simulink model "IRB140"  (R2016b)
settings: Solver=ode113  StartTime=0.0  StopTime=40  RelTol=1e-3
(part 6 of 9)

== matlab function IRB140/Robot2 ==
  data: u input; thetadd output; theta input; thetad input; D output; V output; G output
function [thetadd, D, V, G] = fcn(u, theta, thetad)
theta1 = theta(1);
theta2 = theta(2);
theta3 = theta(3);
theta4 = theta(4);
theta5 = theta(5);
theta6 = theta(6);

qd1 = thetad(1);
qd2 = thetad(2);
qd3 = thetad(3);
qd4 = thetad(4);
qd5 = thetad(5);
qd6 = thetad(6);

g = 9.81;

G1 = 0;
G2 = (g*(57*sin(theta2)*cos(theta3)*cos(theta4)*sin(theta5) + 57*sin(theta3)*cos(theta2)*cos(theta4)*sin(theta5) ...
    + 57*sin(theta2)*sin(theta3)*cos(theta5) + 3186*sin(theta2)*cos(theta3)*sin(theta4) ... 
    + 3186*sin(theta3)*cos(theta2)*sin(theta4) - 57*cos(theta2)*cos(theta3)*cos(theta5) + 418*sin(theta2)*sin(theta3) ... 
    - 418*cos(theta2)*cos(theta3) - 99072*sin(theta2)))/20000;
G3 = 57*(((-cos(theta5) - 22/3)*cos(theta3) + (1062*sin(theta3)*((19*cos(theta4)*sin(theta5))/1062 ...
    + sin(theta4)))/19)*cos(theta2) + ((cos(theta4)*sin(theta5) + (1062*sin(theta4))/19)*cos(theta3) ...
    + (cos(theta5) + 22/3)*sin(theta3))*sin(theta2))*g/20000;
G4 = -57*(sin(theta2)*sin(theta3) - cos(theta2)*cos(theta3))*g*(sin(theta4)*sin(theta5) - (1062*cos(theta4))/19)/20000;
G5 = 57*(cos(theta5)*(sin(theta2)*sin(theta3) - cos(theta2)*cos(theta3))*cos(theta4) ...
    + (cos(theta2)*sin(theta3) + sin(theta2)*cos(theta3))*sin(theta5))*g/20000;
G6 = 0;

G = [G1; G2; G3; G4; G5; G6];

d11 = (19271109*cos(2*theta5))/8000000000 - (386153977*cos(2*theta4))/8000000000 - (295248399*cos(2*theta2))/400000000 - (814991*cos(2*theta6))/2000000000 + (8551647*sin(2*theta2))/200000000 + (510879*sin(2*theta4))/1000000000 + (5043*sin(2*theta5))/500000000 - (1083*cos(theta5))/1000000 - (10836*sin(theta2))/15625 - (1881*sin(theta3))/250000 - (1463*cos(theta2)*cos(theta3))/500000 - (14337*cos(theta3)*sin(theta4))/250000 - (513*cos(theta5)*sin(theta3))/500000 + (1463*sin(theta2)*sin(theta3))/500000 + (1881*cos(2*theta2)*sin(theta3))/250000 + (1881*sin(2*theta2)*cos(theta3))/250000 - (46480089*sin(2*theta4)*cos(theta5))/2000000000 - (2310763*sin(2*theta5)*cos(theta6))/1000000000 + (63931*sin(2*theta4)*sin(theta5))/2000000000 + (3685180549*cos(2*theta2)*cos(2*theta3))/8000000000 - (19271109*cos(2*theta4)*cos(2*theta5))/8000000000 - (2444973*cos(2*theta4)*cos(2*theta6))/2000000000 + (814991*cos(2*theta5)*cos(2*theta6))/2000000000 - (2389617*cos(2*theta2)*sin(2*theta3))/1000000000 - (2389617*cos(2*theta3)*sin(2*theta2))/1000000000 - (5043*cos(2*theta4)*sin(2*theta5))/500000000 - (3685180549*sin(2*theta2)*sin(2*theta3))/8000000000 - (386153977*cos(2*theta2)*cos(2*theta3)*cos(2*theta4))/8000000000 - (57813327*cos(2*theta2)*cos(2*theta3)*cos(2*theta5))/8000000000 + (2444973*cos(2*theta2)*cos(2*theta3)*cos(2*theta6))/2000000000 - (814991*cos(2*theta4)*cos(2*theta5)*cos(2*theta6))/2000000000 + (11151*cos(theta2)*sin(theta3)*sin(theta4))/500000 + (11151*cos(theta3)*sin(theta2)*sin(theta4))/500000 + (399*cos(theta5)*sin(theta2)*sin(theta3))/1000000 + (510879*cos(2*theta2)*cos(2*theta3)*sin(2*theta4))/1000000000 - (15129*cos(2*theta2)*cos(2*theta3)*sin(2*theta5))/500000000 + (386153977*cos(2*theta4)*sin(2*theta2)*sin(2*theta3))/8000000000 + (57813327*cos(2*theta5)*sin(2*theta2)*sin(2*theta3))/8000000000 - (2444973*cos(2*theta6)*sin(2*theta2)*sin(2*theta3))/2000000000 - (510879*sin(2*theta2)*sin(2*theta3)*sin(2*theta4))/1000000000 + (15129*sin(2*theta2)*sin(2*theta3)*sin(2*theta5))/500000000 + (14337*cos(2*theta2)*cos(theta3)*sin(theta4))/250000 + (513*cos(2*theta2)*cos(theta5)*sin(theta3))/500000 + (513*sin(2*theta2)*cos(theta3)*cos(theta5))/500000 - (14337*sin(2*theta2)*sin(theta3)*sin(theta4))/250000 - (2310763*sin(2*theta4)*sin(theta5)*sin(theta6))/500000000 - (1083*cos(2*theta2)*cos(2*theta3)*cos(theta5))/1000000 + (240014043*cos(2*theta2)*sin(2*theta3)*cos(theta4))/500000000 + (240014043*cos(2*theta3)*sin(2*theta2)*cos(theta4))/500000000 + (2310763*cos(2*theta4)*sin(2*theta5)*cos(theta6))/1000000000 + (58876307*cos(2*theta2)*sin(2*theta3)*sin(theta4))/1000000000 + (58876307*cos(2*theta3)*sin(2*theta2)*sin(theta4))/1000000000 + (1083*sin(2*theta2)*sin(2*theta3)*cos(theta5))/1000000 + (814991*sin(2*theta4)*sin(2*theta6)*cos(theta5))/500000000 - (399*cos(theta2)*cos(theta3)*cos(theta5))/1000000 - (513*cos(theta3)*cos(theta4)*sin(theta5))/500000 + (46480089*sin(2*theta2)*sin(2*theta3)*sin(2*theta4)*cos(theta5))/2000000000 - (6932289*sin(2*theta2)*sin(2*theta3)*sin(2*theta5)*cos(theta6))/1000000000 - (63931*sin(2*theta2)*sin(2*theta3)*sin(2*theta4)*sin(theta5))/2000000000 + (513*cos(2*theta2)*cos(theta3)*cos(theta4)*sin(theta5))/500000 - (19271109*cos(2*theta2)*cos(2*theta3)*cos(2*theta4)*cos(2*theta5))/8000000000 - (2444973*cos(2*theta2)*cos(2*theta3)*cos(2*theta4)*cos(2*theta6))/2000000000 - (2444973*cos(2*theta2)*cos(2*theta3)*cos(2*theta5)*cos(2*theta6))/2000000000 - (5043*cos(2*theta2)*cos(2*theta3)*cos(2*theta4)*sin(2*theta5))/500000000 - (513*sin(2*theta2)*cos(theta4)*sin(theta3)*sin(theta5))/500000 + (19271109*cos(2*theta4)*cos(2*theta5)*sin(2*theta2)*sin(2*theta3))/8000000000 + (2444973*cos(2*theta4)*cos(2*theta6)*sin(2*theta2)*sin(2*theta3))/2000000000 + (2444973*cos(2*theta5)*cos(2*theta6)*sin(2*theta2)*sin(2*theta3))/2000000000 + (5043*cos(2*theta4)*sin(2*theta2)*sin(2*theta3)*sin(2*theta5))/500000000 + (1083*cos(2*theta2)*sin(2*theta3)*cos(theta4)*sin(theta5))/1000000 + (63931*cos(2*theta2)*sin(2*theta3)*cos(theta5)*sin(theta4))/1000000000 + (1083*cos(2*theta3)*sin(2*theta2)*cos(theta4)*sin(theta5))/1000000 + (63931*cos(2*theta3)*sin(2*theta2)*cos(theta5)*sin(theta4))/1000000000 + (46480089*cos(2*theta2)*sin(2*theta3)*sin(theta4)*sin(theta5))/1000000000 + (46480089*cos(2*theta3)*sin(2*theta2)*sin(theta4)*sin(theta5))/1000000000 + (399*cos(theta2)*cos(theta4)*sin(theta3)*sin(theta5))/1000000 + (399*cos(theta3)*cos(theta4)*sin(theta2)*sin(theta5))/1000000 - (46480089*cos(2*theta2)*cos(2*theta3)*sin(2*theta4)*cos(theta5))/2000000000 - (5043*cos(2*theta2)*cos(2*theta5)*sin(2*theta3)*cos(theta4))/125000000 - (5043*cos(2*theta3)*cos(2*theta5)*sin(2*theta2)*cos(theta4))/125000000 + (6932289*cos(2*theta2)*cos(2*theta3)*sin(2*theta5)*cos(theta6))/1000000000 + (63931*cos(2*theta2)*cos(2*theta3)*sin(2*theta4)*sin(theta5))/2000000000 + (19271109*cos(2*theta2)*sin(2*theta3)*sin(2*theta5)*cos(theta4))/2000000000 + (19271109*cos(2*theta3)*sin(2*theta2)*sin(2*theta5)*cos(theta4))/2000000000 + (2310763*sin(2*theta2)*sin(2*theta3)*sin(2*theta4)*sin(theta5)*sin(theta6))/500000000 + (2310763*cos(2*theta2)*cos(2*theta3)*cos(2*theta4)*sin(2*theta5)*cos(theta6))/1000000000 + (814991*cos(2*theta2)*cos(2*theta3)*sin(2*theta4)*sin(2*theta6)*cos(theta5))/500000000 + (814991*cos(2*theta2)*cos(2*theta6)*sin(2*theta3)*sin(2*theta5)*cos(theta4))/500000000 + (814991*cos(2*theta3)*cos(2*theta6)*sin(2*theta2)*sin(2*theta5)*cos(theta4))/500000000 - (2310763*cos(2*theta4)*sin(2*theta2)*sin(2*theta3)*sin(2*theta5)*cos(theta6))/1000000000 - (814991*sin(2*theta2)*sin(2*theta3)*sin(2*theta4)*sin(2*theta6)*cos(theta5))/500000000 - (814991*cos(2*theta2)*cos(2*theta3)*cos(2*theta4)*cos(2*theta5)*cos(2*theta6))/2000000000 - (2310763*cos(2*theta2)*sin(2*theta3)*cos(theta5)*sin(theta4)*sin(theta6))/250000000 - (2310763*cos(2*theta3)*sin(2*theta2)*cos(theta5)*sin(theta4)*sin(theta6))/250000000 + (814991*cos(2*theta4)*cos(2*theta5)*cos(2*theta6)*sin(2*theta2)*sin(2*theta3))/2000000000 + (2310763*cos(2*theta2)*cos(2*theta5)*sin(2*theta3)*cos(theta4)*cos(theta6))/250000000 + (2310763*cos(2*theta3)*cos(2*theta5)*sin(2*theta2)*cos(theta4)*cos(theta6))/250000000 - (2310763*cos(2*theta2)*cos(2*theta3)*sin(2*theta4)*sin(theta5)*sin(theta6))/500000000 - (814991*cos(2*theta2)*sin(2*theta3)*sin(2*theta6)*sin(theta4)*sin(theta5))/250000000 - (814991*cos(2*theta3)*sin(2*theta2)*sin(2*theta6)*sin(theta4)*sin(theta5))/250000000 + 5464689505123557/562949953421312;
d12 = (cos(theta4)*(6519928*sin(theta2)*(cos(theta3)*(sin(theta5)*(cos(theta6)*sin(theta6) - 2006614485433615/281474976710656) + cos(theta5)*((2310763*sin(theta6))/1629982 - 5652472290416423/576460752303423488) - 2541777630310401/281474976710656) + sin(theta3)*sin(theta4)*(cos(theta6)^2 + cos(theta5)^2*(cos(theta6)^2 + 1382449826435487/562949953421312) - (cos(theta5)*sin(theta5)*(2310763*cos(theta6) - 5677913230207352589/562949953421312))/814991 + 7778701708353491/281474976710656)) - cos(theta2)*(cos(theta3)*sin(theta4)*(6519928*cos(theta6)^2 + 6519928*cos(theta5)^2*(cos(theta6)^2 + 1382449826435487/562949953421312) - 8*cos(theta5)*sin(theta5)*(2310763*cos(theta6) - 5677913230207352589/562949953421312) + 6339571883992719983581/35184372088832) - sin(theta3)*(sin(theta5)*(6519928*cos(theta6)*sin(theta6) - 46480089) + cos(theta5)*(9243052*sin(theta6) - 63931) - 58876307) + 57348000)))/1000000000 + (cos(theta2)*(1026000*sin(theta4)*sin(theta5) + sin(theta3)*(sin(theta4)*(1083000*sin(theta5) - 9243052*cos(theta6) + 480068430) + cos(theta5)^2*sin(theta4)*(18486104*cos(theta6) - 80688) + 6519928*cos(theta5)*sin(theta4)*sin(theta5)*(cos(theta6)^2 + 1382449826435487/562949953421312) - 42223519) + cos(theta3)*(cos(theta5)*(6519928*cos(theta6)*sin(theta6) - 46480089) - sin(theta5)*(9243052*sin(theta6) - 63931) + 507265041) + 253228718))/1000000000 + (814991*sin(theta2)*(cos(theta3)*(sin(theta4)*((135375*sin(theta5))/814991 - (2310763*cos(theta6))/1629982 + 1295329202195285/17592186044416) + (cos(theta5)^2*sin(theta4)*(2310763*cos(theta6) - 5677913230207352589/562949953421312))/814991 + cos(theta5)*sin(theta4)*sin(theta5)*(cos(theta6)^2 + 1382449826435487/562949953421312) - 1822852035661581/281474976710656) - sin(theta3)*(cos(theta5)*(cos(theta6)*sin(theta6) - 2006614485433615/281474976710656) - sin(theta5)*((2310763*sin(theta6))/1629982 - 5652472290416423/576460752303423488) + 5474846332720429/70368744177664) + 8711646402000795/140737488355328))/125000000 - (cos(theta4)^2*(cos(theta2)*cos(theta3) - sin(theta2)*sin(theta3))*(814991*cos(theta5)*(cos(theta6)*sin(theta6) - 2006614485433615/281474976710656) - 814991*sin(theta5)*((2310763*sin(theta6))/1629982 - 5652472290416423/576460752303423488) + 4601588948062823461131/36028797018963968))/62500000;
d13 = 814991*((cos(theta6)*sin(theta6) - 46480089/6519928)*cos(theta5) + 510879/3259964 + (-(2310763*sin(theta6))/1629982 + 63931/6519928)*sin(theta5))*(sin(theta2)*sin(theta3) - cos(theta2)*cos(theta3))*cos(theta4)^2/62500000 + (((-6519928*((cos(theta6)^2 + 16011145/6519928)*cos(theta5)^2 - 2310763*(cos(theta6) - 10086/2310763)*sin(theta5)*cos(theta5)/814991 + cos(theta6)^2 + 90090735/3259964)*sin(theta4)*cos(theta3) + ((9243052*sin(theta6) - 63931)*cos(theta5) - 58876307 + (6519928*cos(theta6)*sin(theta6) - 46480089)*sin(theta5))*sin(theta3))*cos(theta2) + 6519928*sin(theta2)*((((2310763*sin(theta6))/1629982 - 63931/6519928)*cos(theta5) - 58876307/6519928 + (cos(theta6)*sin(theta6) - 46480089/6519928)*sin(theta5))*cos(theta3) + ((cos(theta6)^2 + 16011145/6519928)*cos(theta5)^2 - 2310763*(cos(theta6) - 10086/2310763)*sin(theta5)*cos(theta5)/814991 + cos(theta6)^2 + 90090735/3259964)*sin(theta4)*sin(theta3)))*cos(theta4))/1000000000 + ((((6519928*cos(theta6)*sin(theta6) - 46480089)*cos(theta5) + 507265041 + (-9243052*sin(theta6) + 63931)*sin(theta5))*cos(theta3) + 6519928*sin(theta3)*(2310763*(cos(theta6) - 10086/2310763)*sin(theta4)*cos(theta5)^2/814991 + sin(theta5)*(cos(theta6)^2 + 16011145/6519928)*sin(theta4)*cos(theta5) - 42223519/6519928 + (-(2310763*cos(theta6))/1629982 + (135375*sin(theta5))/814991 + 240034215/3259964)*sin(theta4)))*cos(theta2))/1000000000 + (814991*sin(theta2)*((2310763*(cos(theta6) - 10086/2310763)*sin(theta4)*cos(theta5)^2/814991 + sin(theta5)*(cos(theta6)^2 + 16011145/6519928)*sin(theta4)*cos(theta5) - 42223519/6519928 + (-(2310763*cos(theta6))/1629982 + (135375*sin(theta5))/814991 + 240034215/3259964)*sin(theta4))*cos(theta3) - ((cos(theta6)*sin(theta6) - 46480089/6519928)*cos(theta5) + 507265041/6519928 + (-(2310763*sin(theta6))/1629982 + 63931/6519928)*sin(theta5))*sin(theta3)))/125000000;
d14 = ((((6519928*cos(theta6)^2 + 16011145)*cos(theta3) - 18486104*cos(theta4)*sin(theta3)*(cos(theta6) - 10086/2310763))*sin(theta2) + 6519928*((2310763*cos(theta4)*(cos(theta6) - 10086/2310763)*cos(theta3))/814991 + sin(theta3)*(cos(theta6)^2 + 16011145/6519928))*cos(theta2))*cos(theta5)^2)/1000000000 + ((((-18486104*cos(theta6) + 80688)*sin(theta5)*cos(theta3) - 6519928*(sin(theta5)*(cos(theta6)^2 + 16011145/6519928)*cos(theta4) - 2310763*(sin(theta6) - 9133/1320436)*sin(theta4)/1629982)*sin(theta3))*sin(theta2) + 6519928*((sin(theta5)*(cos(theta6)^2 + 16011145/6519928)*cos(theta4) - 2310763*(sin(theta6) - 9133/1320436)*sin(theta4)/1629982)*cos(theta3) - (2310763*sin(theta5)*sin(theta3)*(cos(theta6) - 10086/2310763))/814991)*cos(theta2))*cos(theta5))/1000000000 + (((-6519928*cos(theta6)^2 + 373877597)*cos(theta3) + ((9243052*cos(theta6) - 1083000*sin(theta5) - 480068430)*cos(theta4) + (6519928*cos(theta6)*sin(theta4)*sin(theta6) - 46480089*sin(theta4))*sin(theta5) - 58876307*sin(theta4))*sin(theta3) - 1026000*cos(theta4)*sin(theta5) - 57348000*sin(theta4))*sin(theta2))/1000000000 + ((((-9243052*cos(theta6) + 1083000*sin(theta5) + 480068430)*cos(theta4) + (-6519928*cos(theta6)*sin(theta4)*sin(theta6) + 46480089*sin(theta4))*sin(theta5) + 58876307*sin(theta4))*cos(theta3) + (-6519928*cos(theta6)^2 + 373877597)*sin(theta3))*cos(theta2))/1000000000 + (399*cos(theta4)*sin(theta5))/2000000 + (11151*sin(theta4))/1000000;
d15 = ((((9243052*sin(theta6) - 63931)*cos(theta3) + (6519928*cos(theta6)*sin(theta6)*cos(theta4) - 1083000*sin(theta4) - 46480089*cos(theta4))*sin(theta3) - 1026000*sin(theta4))*sin(theta2) + ((-6519928*cos(theta6)*sin(theta6)*cos(theta4) + 1083000*sin(theta4) + 46480089*cos(theta4))*cos(theta3) + (9243052*sin(theta6) - 63931)*sin(theta3))*cos(theta2) + 199500*sin(theta4))*cos(theta5))/1000000000 + ((sin(theta5)*(6519928*cos(theta6)*sin(theta6) - 46480089)*cos(theta3) + 6519928*(-2310763*(sin(theta6) - 9133/1320436)*sin(theta5)*cos(theta4)/1629982 + sin(theta4)*(cos(theta6)^2 + 21347091/3259964))*sin(theta3))*sin(theta2))/1000000000 - 814991*((-2310763*(sin(theta6) - 9133/1320436)*sin(theta5)*cos(theta4)/1629982 + sin(theta4)*(cos(theta6)^2 + 21347091/3259964))*cos(theta3) - (cos(theta6)*sin(theta6) - 46480089/6519928)*sin(theta5)*sin(theta3))*cos(theta2)/125000000;
d16 = ((((2310763*cos(theta6)*cos(theta5) + 1631507*sin(theta5))*cos(theta4) - 2310763*sin(theta4)*sin(theta6))*cos(theta3) + (-2310763*sin(theta5)*cos(theta6) + 1631507*cos(theta5))*sin(theta3))*cos(theta2))/250000000 - (2310763*sin(theta2)*((sin(theta5)*cos(theta6) - (1631507*cos(theta5))/2310763)*cos(theta3) + ((cos(theta6)*cos(theta5) + (1631507*sin(theta5))/2310763)*cos(theta4) - sin(theta4)*sin(theta6))*sin(theta3)))/250000000;
d22 = (((6519928*cos(theta6)^2 + 16011145)*cos(theta5)^2 + (-18486104*cos(theta6) + 80688)*sin(theta5)*cos(theta5) + 6519928*cos(theta6)^2 + 180181470)*cos(theta4)^2)/1000000000 + (((-13039856*cos(theta6)*sin(theta4)*sin(theta6) + 92960178*sin(theta4))*cos(theta5) + ((18486104*sin(theta6) - 127862)*sin(theta4) - 2052000*cos(theta3))*sin(theta5) - 2043516*sin(theta4))*cos(theta4))/1000000000 + ((-6519928*cos(theta6)^2 - 16011145)*cos(theta5)^2)/1000000000 + (((18486104*cos(theta6) - 80688)*sin(theta5) - 2052000*sin(theta3) - 2166000)*cos(theta5))/1000000000 - (14337*sin(theta4)*cos(theta3))/125000 - (1881*sin(theta3))/125000 + 3166244353/1000000000;
d23 = (((6519928*cos(theta6)^2 + 16011145)*cos(theta5)^2 + (-18486104*cos(theta6) + 80688)*sin(theta5)*cos(theta5) + 6519928*cos(theta6)^2 + 180181470)*cos(theta4)^2)/1000000000 + (((-13039856*cos(theta6)*sin(theta4)*sin(theta6) + 92960178*sin(theta4))*cos(theta5) + ((18486104*sin(theta6) - 127862)*sin(theta4) - 1026000*cos(theta3))*sin(theta5) - 2043516*sin(theta4))*cos(theta4))/1000000000 + ((-6519928*cos(theta6)^2 - 16011145)*cos(theta5)^2)/1000000000 + (((18486104*cos(theta6) - 80688)*sin(theta5) - 1026000*sin(theta3) - 2166000)*cos(theta5))/1000000000 - (14337*sin(theta4)*cos(theta3))/250000 - (1881*sin(theta3))/250000 + 37281291/25000000;
d24 = (((18486104*cos(theta6) - 80688)*cos(theta5)^2 + sin(theta5)*(6519928*cos(theta6)^2 + 16011145)*cos(theta5) + (1026000*sin(theta3) + 1083000)*sin(theta5) - 9243052*cos(theta6) + 480068430)*sin(theta4))/1000000000 + (((9243052*sin(theta6) - 63931)*cos(theta5) + (6519928*cos(theta6)*sin(theta6) - 46480089)*sin(theta5) - 57348000*sin(theta3) - 58876307)*cos(theta4))/1000000000;
d25 = (((-1026000*sin(theta3) - 1083000)*cos(theta5) + 6519928*cos(theta6)^2 + 42694182)*cos(theta4))/1000000000 + ((-6519928*cos(theta6)*sin(theta6) + 46480089)*sin(theta4)*cos(theta5))/1000000000 + (2310763*sin(theta5)*((sin(theta6) - 9133/1320436)*sin(theta4) - (256500*cos(theta3))/2310763))/250000000;
d26 = ((2310763*cos(theta6)*cos(theta5) + 1631507*sin(theta5))*sin(theta4))/250000000 + (2310763*sin(theta6)*cos(theta4))/250000000;
d33 = (((6519928*cos(theta6)^2 + 16011145)*cos(theta5)^2 + (-18486104*sin(theta5)*cos(theta6) + 80688*sin(theta5))*cos(theta5) + 6519928*cos(theta6)^2 + 180181470)*cos(theta4)^2)/1000000000 + (((-13039856*cos(theta6)*sin(theta4)*sin(theta6) + 92960178*sin(theta4))*cos(theta5) + (18486104*sin(theta6) - 127862)*sin(theta4)*sin(theta5) - 2043516*sin(theta4))*cos(theta4))/1000000000 + 37281291/25000000 + ((-6519928*cos(theta6)^2 - 16011145)*cos(theta5)^2)/1000000000 + ((18486104*sin(theta5)*cos(theta6) - 80688*sin(theta5) - 2166000)*cos(theta5))/1000000000;
d34 = (((18486104*cos(theta6) - 80688)*cos(theta5)^2 + sin(theta5)*(6519928*cos(theta6)^2 + 16011145)*cos(theta5) - 9243052*cos(theta6) + 1083000*sin(theta5) + 480068430)*sin(theta4))/1000000000 + ((9243052*sin(theta6) - 63931)*cos(theta4)*cos(theta5))/1000000000 + cos(theta4)*(6519928*sin(theta5)*cos(theta6)*sin(theta6) - 46480089*sin(theta5) - 58876307)/1000000000;
d35 = ((-6519928*cos(theta5)*cos(theta6)*sin(theta6) + 9243052*sin(theta6)*sin(theta5) + 46480089*cos(theta5) - 63931*sin(theta5))*sin(theta4))/1000000000 + ((6519928*cos(theta6)^2 - 1083000*cos(theta5) + 42694182)*cos(theta4))/1000000000;
d36 = ((2310763*cos(theta6)*cos(theta5) + 1631507*sin(theta5))*sin(theta4))/250000000 + (2310763*sin(theta6)*cos(theta4))/250000000;
d44 = ((6519928*cos(theta6)^2 + 16011145)*cos(theta5)^2)/1000000000 + ((-18486104*sin(theta5)*cos(theta6) + 80688*sin(theta5))*cos(theta5))/1000000000 - (814991*cos(theta6)^2)/125000000 + 373877597/1000000000;
d45 = ((6519928*sin(theta5)*cos(theta6) + 9243052*cos(theta5))*sin(theta6))/1000000000 - (63931*cos(theta5))/1000000000 - (46480089*sin(theta5))/1000000000;
d46 = (1631507*cos(theta5))/250000000 - (2310763*sin(theta5)*cos(theta6))/250000000;
d55 = (814991*cos(theta6)^2)/125000000 + 21347091/500000000;
d56 = (2310763*sin(theta6))/250000000;
d66 = 1631507/250000000;

D = [d11 d12 d13 d14 d15 d16; d12 d22 d23 d24 d25 d26; d13 d23 d33 d34 d35 d36; d14 d24 d34 d44 d45 d46; d15 d25 d35 d45 d55 d56; d16 d26 d36 d46 d56 d66];

v1 = (814991*qd1*((((((2310763*qd5)/814991 + qd6*sin(theta6))*cos(theta6) - (10086*qd5)/814991)*cos(theta5)^2 + (((16011145*qd5)/6519928 + qd5*cos(theta6)^2 - (2310763*qd6*sin(theta6))/1629982)*sin(theta5) + 2*qd4*sin(theta6)*cos(theta6) - (46480089*qd4)/3259964)*cos(theta5) - 2310763*(-9133/1320436 + sin(theta6))*qd4*sin(theta5)/814991 + (qd6*sin(theta6) - (2310763*qd5)/1629982)*cos(theta6) + (5043*qd5)/814991 + (510879*qd4)/1629982)*cos(theta4)^2 + ((qd4*(16011145/6519928 + cos(theta6)^2)*sin(theta4) + 4621526*(cos(theta6) - 10086/2310763)*(qd2 + qd3)/814991)*cos(theta5)^2 + ((-2310763*(cos(theta6) - 10086/2310763)*qd4*sin(theta4)/814991 + 2*(16011145/6519928 + cos(theta6)^2)*(qd2 + qd3))*sin(theta5) + 2*(qd6*cos(theta6)^2 - (2310763*qd5*sin(theta6))/3259964 + (63931*qd5)/13039856 - qd6/2)*sin(theta4))*cos(theta5) + (((-qd5*sin(theta6) - (2310763*qd6)/1629982)*cos(theta6) + (46480089*qd5)/6519928)*sin(theta4) + (270750*qd2)/814991 + (270750*qd3)/814991)*sin(theta5) + qd4*(cos(theta6)^2 + 90090735/3259964)*sin(theta4) - 2310763*(cos(theta6) - 240034215/4621526)*(qd2 + qd3)/814991)*cos(theta4) + (((2310763*qd5)/814991 + qd6*sin(theta6))*cos(theta6) - (10086*qd5)/814991)*cos(theta5)^2 + (((16011145*qd5)/6519928 + qd5*cos(theta6)^2 - (2310763*qd6*sin(theta6))/1629982)*sin(theta5) - 2310763*(-9133/1320436 + sin(theta6))*(qd2 + qd3)*sin(theta4)/814991 - qd4*sin(theta6)*cos(theta6) + (46480089*qd4)/6519928)*cos(theta5) + (-2*(sin(theta6)*cos(theta6) - 46480089/6519928)*(qd2 + qd3)*sin(theta4) - (63931*qd4)/6519928 + (135375*qd5)/814991 + (2310763*sin(theta6)*qd4)/1629982)*sin(theta5) + ((58876307*qd2)/3259964 + (58876307*qd3)/3259964)*sin(theta4) + (-(2310763*qd5)/1629982 - 2*qd6*sin(theta6))*cos(theta6) + (5043*qd5)/814991 - (2389617*qd3)/3259964 - (510879*qd4)/3259964 - (2389617*qd2)/3259964)*cos(theta3)^2 + (sin(theta3)*((16011145/6519928 + cos(theta6)^2)*cos(theta5)^2 - 2310763*(cos(theta6) - 10086/2310763)*sin(theta5)*cos(theta5)/814991 + cos(theta6)^2 + 90090735/3259964)*(qd2 + qd3)*cos(theta4)^2 + (2*((16011145*qd5)/6519928 + qd5*cos(theta6)^2 - (2310763*qd6*sin(theta6))/1629982)*sin(theta3)*cos(theta5)^2 + ((((-2*qd6*sin(theta6) - (4621526*qd5)/814991)*cos(theta6) + (20172*qd5)/814991)*sin(theta5) - 2*(sin(theta6)*cos(theta6) - 46480089/6519928)*(qd2 + qd3)*sin(theta4) - (2310763*sin(theta6)*qd4)/1629982 + (63931*qd4)/6519928 + (135375*qd5)/814991)*sin(theta3) + (64125*qd5)/814991)*cos(theta5) + ((2310763*(-9133/1320436 + sin(theta6))*(qd2 + qd3)*sin(theta4)/814991 - qd4*sin(theta6)*cos(theta6) + (46480089*qd4)/6519928)*sin(theta5) + (-(510879*qd3)/1629982 - (510879*qd2)/1629982)*sin(theta4) - (16011145*qd5)/6519928 + (58876307*qd4)/6519928 - qd5*cos(theta6)^2 + (2310763*qd6*sin(theta6))/1629982)*sin(theta3) + (3584250*qd4)/814991)*cos(theta4) + (-2310763*(cos(theta6) - 10086/2310763)*qd4*sin(theta4)/814991 + (16011145/6519928 + cos(theta6)^2)*(qd2 + qd3))*sin(theta3)*cos(theta5)^2 + ((((-(16011145*qd4)/6519928 - qd4*cos(theta6)^2)*sin(theta4) - 2310763*(cos(theta6) - 10086/2310763)*(qd2 + qd3)/814991)*sin(theta5) + ((-qd5*sin(theta6) - (2310763*qd6)/1629982)*cos(theta6) + (46480089*qd5)/6519928)*sin(theta4) + (270750*qd2)/814991 + (270750*qd3)/814991)*sin(theta3) + (64125*qd3)/814991 + (128250*qd2)/814991)*cos(theta5) + (-2*(qd6*cos(theta6)^2 - (2310763*qd5*sin(theta6))/3259964 + (135375*qd4)/1629982 + (63931*qd5)/13039856 - qd6/2)*sin(theta4)*sin(theta5) + 2310763*(cos(theta6) - 240034215/4621526)*qd4*sin(theta4)/1629982 - 2*(qd2 + qd3)*(cos(theta6)^2 + 510474629/6519928))*sin(theta3) + (470250*qd3)/814991 - (64125*qd4*sin(theta5)*sin(theta4))/814991 + (940500*qd2)/814991)*cos(theta3) + (((-(2310763*qd5)/1629982 - qd6*sin(theta6)/2)*cos(theta6) + (5043*qd5)/814991)*cos(theta5)^2 + ((-(16011145*qd5)/13039856 - qd5*cos(theta6)^2/2 + (2310763*qd6*sin(theta6))/3259964)*sin(theta5) - qd4*sin(theta6)*cos(theta6) + (46480089*qd4)/6519928)*cos(theta5) + 2310763*(-9133/1320436 + sin(theta6))*qd4*sin(theta5)/1629982 + (-qd6*sin(theta6)/2 + (2310763*qd5)/3259964)*cos(theta6) - (5043*qd5)/1629982 - (510879*qd4)/3259964)*cos(theta4)^2 + (((-(16011145*qd4)/13039856 - qd4*cos(theta6)^2/2)*sin(theta4) - 2310763*(cos(theta6) - 10086/2310763)*(qd2 + qd3)/814991)*cos(theta5)^2 + ((2310763*(cos(theta6) - 10086/2310763)*qd4*sin(theta4)/1629982 - (16011145/6519928 + cos(theta6)^2)*(qd2 + qd3))*sin(theta5) - (qd6*cos(theta6)^2 - (2310763*qd5*sin(theta6))/3259964 + (63931*qd5)/13039856 - qd6/2)*sin(theta4))*cos(theta5) - 128250*(qd2 + qd3/2)*sin(theta5)*sin(theta3)/814991 + (((qd5*sin(theta6)/2 + (2310763*qd6)/3259964)*cos(theta6) - (46480089*qd5)/13039856)*sin(theta4) - (135375*qd2)/814991 - (135375*qd3)/814991)*sin(theta5) + (-qd4*cos(theta6)^2/2 - (90090735*qd4)/6519928)*sin(theta4) + 2310763*(cos(theta6) - 240034215/4621526)*(qd2 + qd3)/1629982)*cos(theta4) + ((-(2310763*qd5)/1629982 - qd6*sin(theta6)/2)*cos(theta6) + (5043*qd5)/814991)*cos(theta5)^2 + ((-(16011145*qd5)/13039856 - qd5*cos(theta6)^2/2 + (2310763*qd6*sin(theta6))/3259964)*sin(theta5) + 2310763*(-9133/1320436 + sin(theta6))*(qd2 + qd3)*sin(theta4)/1629982 + ((sin(theta6)*cos(theta6) - 46480089/6519928)*qd4)/2)*cos(theta5) + (-(64125*qd5*sin(theta5))/814991 - 7168500*(qd2 + qd3/2)*sin(theta4)/814991)*sin(theta3) + ((sin(theta6)*cos(theta6) - 46480089/6519928)*(qd2 + qd3)*sin(theta4) + (63931*qd4)/13039856 - (135375*qd5)/1629982 - (2310763*sin(theta6)*qd4)/3259964)*sin(theta5) + (-(58876307*qd2)/6519928 - (58876307*qd3)/6519928)*sin(theta4) + ((2310763*qd5)/3259964 + qd6*sin(theta6))*cos(theta6) - (5043*qd5)/1629982 + (2389617*qd3)/6519928 + (510879*qd4)/6519928 + (11286963*qd2)/1629982)*cos(theta2)^2)/31250000 + ((26079712*(((16011145/6519928 + cos(theta6)^2)*cos(theta5)^2 - 2310763*(cos(theta6) - 10086/2310763)*sin(theta5)*cos(theta5)/814991 + cos(theta6)^2 + 90090735/3259964)*(qd2 + qd3)*cos(theta4)^2 + ((-(2310763*qd6*sin(theta6))/814991 + 2*qd5*cos(theta6)^2 + (16011145*qd5)/3259964)*cos(theta5)^2 + (((-2*qd6*sin(theta6) - (4621526*qd5)/814991)*cos(theta6) + (20172*qd5)/814991)*sin(theta5) - 2*(sin(theta6)*cos(theta6) - 46480089/6519928)*(qd2 + qd3)*sin(theta4) - (2310763*sin(theta6)*qd4)/1629982 + (63931*qd4)/6519928 + (135375*qd5)/814991)*cos(theta5) + (2310763*(-9133/1320436 + sin(theta6))*(qd2 + qd3)*sin(theta4)/814991 - qd4*sin(theta6)*cos(theta6) + (46480089*qd4)/6519928)*sin(theta5) + (-(510879*qd3)/1629982 - (510879*qd2)/1629982)*sin(theta4) - (16011145*qd5)/6519928 + (58876307*qd4)/6519928 - qd5*cos(theta6)^2 + (2310763*qd6*sin(theta6))/1629982)*cos(theta4) + (-2310763*(cos(theta6) - 10086/2310763)*qd4*sin(theta4)/814991 + (16011145/6519928 + cos(theta6)^2)*(qd2 + qd3))*cos(theta5)^2 + (((-(16011145*qd4)/6519928 - qd4*cos(theta6)^2)*sin(theta4) - 2310763*(cos(theta6) - 10086/2310763)*(qd2 + qd3)/814991)*sin(theta5) + ((-qd5*sin(theta6) - (2310763*qd6)/1629982)*cos(theta6) + (46480089*qd5)/6519928)*sin(theta4) + (270750*qd2)/814991 + (270750*qd3)/814991)*cos(theta5) - 2*(qd6*cos(theta6)^2 - (2310763*qd5*sin(theta6))/3259964 + (135375*qd4)/1629982 + (63931*qd5)/13039856 - qd6/2)*sin(theta4)*sin(theta5) + 2310763*(cos(theta6) - 240034215/4621526)*qd4*sin(theta4)/1629982 - 2*(qd2 + qd3)*(cos(theta6)^2 + 510474629/6519928))*sin(theta2)*qd1*cos(theta3)^2 + (((-26079712*(((2310763*qd5)/814991 + qd6*sin(theta6))*cos(theta6) - (10086*qd5)/814991)*sin(theta3)*qd1*sin(theta2) - 13039856*(16011145/6519928 + cos(theta6)^2)*qd4*(qd2 + qd3))*cos(theta5)^2 + (-26079712*(((16011145*qd5)/6519928 + qd5*cos(theta6)^2 - (2310763*qd6*sin(theta6))/1629982)*sin(theta5) + 2*qd4*sin(theta6)*cos(theta6) - (46480089*qd4)/3259964)*sin(theta3)*qd1*sin(theta2) - 26079712*(-2310763*(cos(theta6) - 10086/2310763)*qd4*sin(theta5)/1629982 + qd6*cos(theta6)^2 - (2310763*qd5*sin(theta6))/3259964 + (63931*qd5)/13039856 - qd6/2)*(qd2 + qd3))*cos(theta5) - 26079712*sin(theta3)*(-2310763*(-9133/1320436 + sin(theta6))*qd4*sin(theta5)/814991 + (qd6*sin(theta6) - (2310763*qd5)/1629982)*cos(theta6) + (5043*qd5)/814991 + (510879*qd4)/1629982)*qd1*sin(theta2) - 13039856*(((-qd5*sin(theta6) - (2310763*qd6)/1629982)*cos(theta6) + (46480089*qd5)/6519928)*sin(theta5) + qd4*(cos(theta6)^2 + 90090735/3259964))*(qd2 + qd3))*cos(theta4)^2 + ((-26079712*(qd4*(16011145/6519928 + cos(theta6)^2)*sin(theta4) + 4621526*(cos(theta6) - 10086/2310763)*(qd2 + qd3)/814991)*sin(theta3)*qd1*sin(theta2) + 13039856*(((2310763*qd5)/814991 + qd6*sin(theta6))*cos(theta6) - (10086*qd5)/814991)*(qd2 + qd3)*sin(theta4) + 13039856*cos(theta6)^2*qd4*qd5 - 18486104*sin(theta6)*qd4*qd6 + 32022290*qd4*qd5)*cos(theta5)^2 + (-52159424*sin(theta3)*qd1*((-2310763*(cos(theta6) - 10086/2310763)*qd4*sin(theta4)/1629982 + (16011145/6519928 + cos(theta6)^2)*(qd2 + qd3))*sin(theta5) + (qd6*cos(theta6)^2 - (2310763*qd5*sin(theta6))/3259964 + (63931*qd5)/13039856 - qd6/2)*sin(theta4))*sin(theta2) + (13039856*((16011145*qd5)/6519928 + qd5*cos(theta6)^2 - (2310763*qd6*sin(theta6))/1629982)*(qd2 + qd3)*sin(theta4) - 13039856*(((2310763*qd5)/814991 + qd6*sin(theta6))*cos(theta6) - (10086*qd5)/814991)*qd4)*sin(theta5) + 26079712*(sin(theta6)*cos(theta6) - 46480089/6519928)*qd4*(qd2 + qd3)*sin(theta4) - 13039856*cos(theta6)^2*qd5*qd6 + (9243052*qd2^2 + 18486104*qd2*qd3 + 9243052*qd3^2 - 9243052*qd4^2 + 9243052*qd5^2 - 9243052*qd6^2)*sin(theta6) - 63931*qd2^2 - 127862*qd2*qd3 - 63931*qd3^2 + 63931*qd4^2 + 2166000*qd4*qd5 - 63931*qd5^2 + 13045956*qd5*qd6)*cos(theta5) - 26079712*(((((-qd5*sin(theta6) - (2310763*qd6)/1629982)*cos(theta6) + (46480089*qd5)/6519928)*sin(theta4) + (270750*qd2)/814991 + (270750*qd3)/814991)*sin(theta5) + qd4*(cos(theta6)^2 + 90090735/3259964)*sin(theta4) - 2310763*(cos(theta6) - 240034215/4621526)*(qd2 + qd3)/814991)*sin(theta3) + 128250*(qd2 + qd3/2)*sin(theta5)/814991)*qd1*sin(theta2) + (-36972208*(-9133/1320436 + sin(theta6))*qd4*(qd2 + qd3)*sin(theta4) + 6519928*sin(theta6)*(qd2^2 + 2*qd2*qd3 + qd3^2 - qd4^2 + qd5^2)*cos(theta6) + (399000*qd2 + 399000*qd3)*qd1 - 46480089*qd2^2 - 92960178*qd2*qd3 - 46480089*qd3^2 + 46480089*qd4^2 - 46480089*qd5^2)*sin(theta5) + 13039856*((qd6*sin(theta6) - (2310763*qd5)/1629982)*cos(theta6) + (5043*qd5)/814991 + (510879*qd4)/1629982)*(qd2 + qd3)*sin(theta4) - 13039856*cos(theta6)^2*qd4*qd5 - 58876307*qd2^2 - 117752614*qd2*qd3 - 58876307*qd3^2 + 58876307*qd4^2 - 58705327*qd4*qd5)*cos(theta4) + (-26079712*(((2310763*qd5)/814991 + qd6*sin(theta6))*cos(theta6) - (10086*qd5)/814991)*sin(theta3)*qd1*sin(theta2) + 18486104*(cos(theta6) - 10086/2310763)*(qd2 + qd3 - qd4)*(qd2 + qd3 + qd4)*sin(theta4) + 13039856*(16011145/6519928 + cos(theta6)^2)*qd4*(qd2 + qd3))*cos(theta5)^2 + (-26079712*sin(theta3)*(((16011145*qd5)/6519928 + qd5*cos(theta6)^2 - (2310763*qd6*sin(theta6))/1629982)*sin(theta5) - 2310763*(-9133/1320436 + sin(theta6))*(qd2 + qd3)*sin(theta4)/814991 - qd4*sin(theta6)*cos(theta6) + (46480089*qd4)/6519928)*qd1*sin(theta2) + (6519928*(16011145/6519928 + cos(theta6)^2)*(qd2 + qd3 - qd4)*(qd2 + qd3 + qd4)*sin(theta4) - 36972208*(cos(theta6) - 10086/2310763)*qd4*(qd2 + qd3))*sin(theta5) + 13039856*qd6*(-(2310763*qd4*cos(theta6)*sin(theta4))/1629982 + (cos(theta6)^2 + 1525/3259964)*(qd2 + qd3)))*cos(theta5) + 52159424*qd1*((((sin(theta6)*cos(theta6) - 46480089/6519928)*(qd2 + qd3)*sin(theta4) + (63931*qd4)/13039856 - (135375*qd5)/1629982 - (2310763*sin(theta6)*qd4)/3259964)*sin(theta5) + (-(58876307*qd2)/6519928 - (58876307*qd3)/6519928)*sin(theta4) + ((2310763*qd5)/3259964 + qd6*sin(theta6))*cos(theta6) - (5043*qd5)/1629982 + (2389617*qd3)/6519928 + (510879*qd4)/6519928 + (2389617*qd2)/6519928)*sin(theta3) - (64125*qd5*sin(theta5))/1629982 - 3584250*(qd2 + qd3/2)*sin(theta4)/814991)*sin(theta2) + ((-13039856*cos(theta6)^2*qd4*qd6 + 1083000*qd2^2 + 2166000*qd2*qd3 + 1083000*qd3^2 - 1083000*qd4^2 - 6100*qd4*qd6 - 1083000*qd5^2)*sin(theta4) - 18486104*qd6*(qd2 + qd3)*cos(theta6) + 399000*qd1*qd5)*sin(theta5) + ((13039856*sin(theta6)*qd5*qd6 - 9243052*qd2^2 - 18486104*qd2*qd3 - 9243052*qd3^2 + 9243052*qd4^2 - 9243052*qd6^2)*cos(theta6) + (22302000*qd2 + 22302000*qd3)*qd1 + 480068430*(qd2 + qd3 + qd4)*(qd2 + qd3 - qd4))*sin(theta4) - 42223519*(qd2 + qd3 - (554059067*qd4)/42223519)*(qd2 + qd3))*cos(theta3) - 13039856*(qd1*sin(theta2)*(16011145/6519928 + cos(theta6)^2)*cos(theta5)^2 + (-2310763*(cos(theta6) - 10086/2310763)*sin(theta5)*qd1*sin(theta2)/814991 - (sin(theta6)*cos(theta6) - 46480089/6519928)*sin(theta3)*(qd2 + qd3))*cos(theta5) + qd1*(cos(theta6)^2 + 90090735/3259964)*sin(theta2) + 2310763*(-510879/4621526 + (-9133/1320436 + sin(theta6))*sin(theta5))*sin(theta3)*(qd2 + qd3)/1629982)*(qd2 + qd3)*cos(theta4)^2 + (((-26079712*qd1*cos(theta6)^2*qd5 + 36972208*qd1*sin(theta6)*qd6 - 64044580*qd1*qd5)*sin(theta2) + 6519928*(16011145/6519928 + cos(theta6)^2)*sin(theta3)*sin(theta4)*(qd2 + qd3)^2)*cos(theta5)^2 + (26079712*qd1*(-(64125*qd5*sin(theta3))/814991 + (((2310763*qd5)/814991 + qd6*sin(theta6))*cos(theta6) - (10086*qd5)/814991)*sin(theta5) + (sin(theta6)*cos(theta6) - 46480089/6519928)*(qd2 + qd3)*sin(theta4) + (2310763*sin(theta6)*qd4)/3259964 - (63931*qd4)/13039856 - (135375*qd5)/1629982)*sin(theta2) + 399000*sin(theta3)*(-330109*(cos(theta6) - 10086/2310763)*sin(theta4)*(qd2 + qd3)^2*sin(theta5)/7125 + qd5*((1629982*sin(theta6)*(qd2 + qd3)*cos(theta6))/49875 + qd1 - (15493363*qd2)/66500 - (15493363*qd3)/66500)))*cos(theta5) + 13039856*(-(7168500*qd4*sin(theta3))/814991 + (-2310763*(-9133/1320436 + sin(theta6))*(qd2 + qd3)*sin(theta4)/814991 + (sin(theta6)*cos(theta6) - 46480089/6519928)*qd4)*sin(theta5) + ((510879*qd3)/1629982 + (510879*qd2)/1629982)*sin(theta4) + (16011145*qd5)/6519928 - (58876307*qd4)/6519928 + qd5*cos(theta6)^2 - (2310763*qd6*sin(theta6))/1629982)*qd1*sin(theta2) + 22302000*sin(theta3)*(814991*(qd6*cos(theta6)^2 - (2310763*qd5*sin(theta6))/1629982 + (63931*qd5)/6519928 - (3261489*qd6)/3259964)*(qd2 + qd3)*sin(theta5)/1393875 + 814991*(cos(theta6)^2 + 90090735/3259964)*(qd2 + qd3)^2*sin(theta4)/2787750 + qd1*qd4))*cos(theta4) + (-13039856*(-2310763*(cos(theta6) - 10086/2310763)*qd4*sin(theta4)/814991 + (16011145/6519928 + cos(theta6)^2)*(qd2 + qd3))*qd1*sin(theta2) + 13039856*sin(theta3)*(((16011145*qd5)/6519928 + qd5*cos(theta6)^2 - (2310763*qd6*sin(theta6))/1629982)*(qd2 + qd3)*sin(theta4) - (((2310763*qd5)/814991 + qd6*sin(theta6))*cos(theta6) - (10086*qd5)/814991)*qd4))*cos(theta5)^2 + (13039856*qd1*((-(256500*qd2)/814991 - (128250*qd3)/814991)*sin(theta3) + (qd4*(16011145/6519928 + cos(theta6)^2)*sin(theta4) + 2310763*(cos(theta6) - 10086/2310763)*(qd2 + qd3)/814991)*sin(theta5) + ((qd5*sin(theta6) + (2310763*qd6)/1629982)*cos(theta6) - (46480089*qd5)/6519928)*sin(theta4) - (270750*qd2)/814991 - (270750*qd3)/814991)*sin(theta2) + 399000*((-1629982*(((2310763*qd5)/814991 + qd6*sin(theta6))*cos(theta6) - (10086*qd5)/814991)*(qd2 + qd3)*sin(theta4)/49875 - 1629982*((16011145*qd5)/6519928 + qd5*cos(theta6)^2 - (2310763*qd6*sin(theta6))/1629982)*qd4/49875)*sin(theta5) - (814991*sin(theta6)*(qd2 + qd3 + qd5)*(qd2 + qd3 - qd5)*cos(theta6))/49875 + (qd2 + qd3)*qd1 + 15493363*(qd2 + qd3 + qd5)*(qd2 + qd3 - qd5)/133000)*sin(theta3))*cos(theta5) + 26079712*(((64125*qd4*sin(theta5)*sin(theta4))/814991 - (940500*qd2)/814991 - (470250*qd3)/814991)*sin(theta3) + (qd6*cos(theta6)^2 - (2310763*qd5*sin(theta6))/3259964 + (135375*qd4)/1629982 + (63931*qd5)/13039856 - qd6/2)*sin(theta4)*sin(theta5) - 2310763*(cos(theta6) - 240034215/4621526)*qd4*sin(theta4)/3259964 + (qd2 + qd3)*cos(theta6)^2 + (2497191253*qd2)/13039856 + (510474629*qd3)/6519928)*qd1*sin(theta2) + ((-399000*qd1*sin(theta4)*qd4 + 13039856*cos(theta6)^2*qd5*qd6 + (9243052*qd2^2 + 18486104*qd2*qd3 + 9243052*qd3^2 - 9243052*qd5^2 + 9243052*qd6^2)*sin(theta6) - 63931*qd2^2 - 127862*qd2*qd3 - 63931*qd3^2 + 63931*qd5^2 - 13045956*qd5*qd6)*sin(theta5) + 18486104*(qd6*sin(theta6) + (26683037*qd5)/18486104)*(qd2 + qd3)*sin(theta4) + (13039856*sin(theta6)*qd4*qd6 + 18486104*qd4*qd5)*cos(theta6) + (2926000*qd2 + 2926000*qd3)*qd1 - 507265041*qd2^2 - 1014530082*qd2*qd3 - 507265041*qd3^2 - 80688*qd4*qd5)*sin(theta3) - 693504000*qd1*qd2 + 403583352*qd2^2)*cos(theta2))/1000000000 - 814991*(((((2310763*qd5)/814991 + qd6*sin(theta6))*cos(theta6) - (10086*qd5)/814991)*cos(theta5)^2 + (((16011145*qd5)/6519928 + qd5*cos(theta6)^2 - (2310763*qd6*sin(theta6))/1629982)*sin(theta5) + 2*qd4*sin(theta6)*cos(theta6) - (46480089*qd4)/3259964)*cos(theta5) - 2310763*(-9133/1320436 + sin(theta6))*qd4*sin(theta5)/814991 + (qd6*sin(theta6) - (2310763*qd5)/1629982)*cos(theta6) + (5043*qd5)/814991 + (510879*qd4)/1629982)*cos(theta4)^2 + ((qd4*(16011145/6519928 + cos(theta6)^2)*sin(theta4) + 4621526*(cos(theta6) - 10086/2310763)*(qd2 + qd3)/814991)*cos(theta5)^2 + ((-2310763*(cos(theta6) - 10086/2310763)*qd4*sin(theta4)/814991 + 2*(16011145/6519928 + cos(theta6)^2)*(qd2 + qd3))*sin(theta5) + 2*(qd6*cos(theta6)^2 - (2310763*qd5*sin(theta6))/3259964 + (63931*qd5)/13039856 - qd6/2)*sin(theta4))*cos(theta5) + (((-qd5*sin(theta6) - (2310763*qd6)/1629982)*cos(theta6) + (46480089*qd5)/6519928)*sin(theta4) + (270750*qd2)/814991 + (270750*qd3)/814991)*sin(theta5) + qd4*(cos(theta6)^2 + 90090735/3259964)*sin(theta4) - 2310763*(cos(theta6) - 240034215/4621526)*(qd2 + qd3)/814991)*cos(theta4) + (((2310763*qd5)/814991 + qd6*sin(theta6))*cos(theta6) - (10086*qd5)/814991)*cos(theta5)^2 + (((16011145*qd5)/6519928 + qd5*cos(theta6)^2 - (2310763*qd6*sin(theta6))/1629982)*sin(theta5) - 2310763*(-9133/1320436 + sin(theta6))*(qd2 + qd3)*sin(theta4)/814991 - qd4*sin(theta6)*cos(theta6) + (46480089*qd4)/6519928)*cos(theta5) + (-2*(sin(theta6)*cos(theta6) - 46480089/6519928)*(qd2 + qd3)*sin(theta4) - (63931*qd4)/6519928 + (135375*qd5)/814991 + (2310763*sin(theta6)*qd4)/1629982)*sin(theta5) + ((58876307*qd2)/3259964 + (58876307*qd3)/3259964)*sin(theta4) + (-(2310763*qd5)/1629982 - 2*qd6*sin(theta6))*cos(theta6) + (5043*qd5)/814991 - (2389617*qd3)/3259964 - (510879*qd4)/3259964 - (2389617*qd2)/3259964)*qd1*cos(theta3)^2/62500000 + ((-13039856*(qd1*sin(theta3)*(16011145/6519928 + cos(theta6)^2)*cos(theta5)^2 + (-(sin(theta6)*cos(theta6) - 46480089/6519928)*(qd2 + qd3)*sin(theta2) - 2310763*(cos(theta6) - 10086/2310763)*sin(theta5)*sin(theta3)*qd1/814991)*cos(theta5) + 2310763*(-510879/4621526 + (-9133/1320436 + sin(theta6))*sin(theta5))*(qd2 + qd3)*sin(theta2)/1629982 + qd1*sin(theta3)*(cos(theta6)^2 + 90090735/3259964))*(qd2 + qd3)*cos(theta4)^2 + ((6519928*(16011145/6519928 + cos(theta6)^2)*sin(theta4)*(qd2 + qd3)^2*sin(theta2) - 26079712*((16011145*qd5)/6519928 + qd5*cos(theta6)^2 - (2310763*qd6*sin(theta6))/1629982)*sin(theta3)*qd1)*cos(theta5)^2 + ((-18486104*(cos(theta6) - 10086/2310763)*sin(theta4)*(qd2 + qd3)^2*sin(theta5) + 399000*qd5*((1629982*sin(theta6)*(qd2 + qd3)*cos(theta6))/49875 + qd1 - (15493363*qd2)/66500 - (15493363*qd3)/66500))*sin(theta2) + 26079712*(((((2310763*qd5)/814991 + qd6*sin(theta6))*cos(theta6) - (10086*qd5)/814991)*sin(theta5) + (sin(theta6)*cos(theta6) - 46480089/6519928)*(qd2 + qd3)*sin(theta4) + (2310763*sin(theta6)*qd4)/3259964 - (63931*qd4)/13039856 - (135375*qd5)/1629982)*sin(theta3) - (64125*qd5)/814991)*qd1)*cos(theta5) + (13039856*(qd6*cos(theta6)^2 - (2310763*qd5*sin(theta6))/1629982 + (63931*qd5)/6519928 - (3261489*qd6)/3259964)*(qd2 + qd3)*sin(theta5) + 6519928*(cos(theta6)^2 + 90090735/3259964)*(qd2 + qd3)^2*sin(theta4) + 22302000*qd1*qd4)*sin(theta2) + 13039856*qd1*(((-2310763*(-9133/1320436 + sin(theta6))*(qd2 + qd3)*sin(theta4)/814991 + (sin(theta6)*cos(theta6) - 46480089/6519928)*qd4)*sin(theta5) + ((510879*qd3)/1629982 + (510879*qd2)/1629982)*sin(theta4) + (16011145*qd5)/6519928 - (58876307*qd4)/6519928 + qd5*cos(theta6)^2 - (2310763*qd6*sin(theta6))/1629982)*sin(theta3) - (7168500*qd4)/814991))*cos(theta4) + ((13039856*((16011145*qd5)/6519928 + qd5*cos(theta6)^2 - (2310763*qd6*sin(theta6))/1629982)*(qd2 + qd3)*sin(theta4) - 13039856*(((2310763*qd5)/814991 + qd6*sin(theta6))*cos(theta6) - (10086*qd5)/814991)*qd4)*sin(theta2) - 13039856*(-2310763*(cos(theta6) - 10086/2310763)*qd4*sin(theta4)/814991 + (16011145/6519928 + cos(theta6)^2)*(qd2 + qd3))*sin(theta3)*qd1)*cos(theta5)^2 + (((-13039856*(((2310763*qd5)/814991 + qd6*sin(theta6))*cos(theta6) - (10086*qd5)/814991)*(qd2 + qd3)*sin(theta4) - 13039856*cos(theta6)^2*qd4*qd5 + 18486104*sin(theta6)*qd4*qd6 - 32022290*qd4*qd5)*sin(theta5) - 6519928*sin(theta6)*(qd2 + qd3 + qd5)*(qd2 + qd3 - qd5)*cos(theta6) + (399000*qd2 + 399000*qd3)*qd1 + 46480089*(qd2 + qd3 + qd5)*(qd2 + qd3 - qd5))*sin(theta2) + 13039856*qd1*(((qd4*(16011145/6519928 + cos(theta6)^2)*sin(theta4) + 2310763*(cos(theta6) - 10086/2310763)*(qd2 + qd3)/814991)*sin(theta5) + ((qd5*sin(theta6) + (2310763*qd6)/1629982)*cos(theta6) - (46480089*qd5)/6519928)*sin(theta4) - (270750*qd2)/814991 - (270750*qd3)/814991)*sin(theta3) - (128250*qd2)/814991 - (128250*qd3)/814991))*cos(theta5) + ((-399000*qd1*sin(theta4)*qd4 + 13039856*cos(theta6)^2*qd5*qd6 + (9243052*qd2^2 + 18486104*qd2*qd3 + 9243052*qd3^2 - 9243052*qd5^2 + 9243052*qd6^2)*sin(theta6) - 63931*qd2^2 - 127862*qd2*qd3 - 63931*qd3^2 + 63931*qd5^2 - 13045956*qd5*qd6)*sin(theta5) + 18486104*(qd6*sin(theta6) + (26683037*qd5)/18486104)*(qd2 + qd3)*sin(theta4) + (13039856*sin(theta6)*qd4*qd6 + 18486104*qd4*qd5)*cos(theta6) + (2926000*qd2 + 2926000*qd3)*qd1 - 507265041*qd2^2 - 1014530082*qd2*qd3 - 507265041*qd3^2 - 80688*qd4*qd5)*sin(theta2) + 26079712*(((qd6*cos(theta6)^2 - (2310763*qd5*sin(theta6))/3259964 + (135375*qd4)/1629982 + (63931*qd5)/13039856 - qd6/2)*sin(theta4)*sin(theta5) - 2310763*(cos(theta6) - 240034215/4621526)*qd4*sin(theta4)/3259964 + (qd2 + qd3)*(cos(theta6)^2 + 510474629/6519928))*sin(theta3) + (64125*qd4*sin(theta5)*sin(theta4))/814991 - (470250*qd2)/814991 - (470250*qd3)/814991)*qd1)*cos(theta3))/1000000000 + (((13039856*(16011145/6519928 + cos(theta6)^2)*qd4*sin(theta3)*(qd2 + qd3)*sin(theta2) + 13039856*(((2310763*qd5)/814991 + qd6*sin(theta6))*cos(theta6) - (10086*qd5)/814991)*qd1)*cos(theta5)^2 + (26079712*(-2310763*(cos(theta6) - 10086/2310763)*qd4*sin(theta5)/1629982 + qd6*cos(theta6)^2 - (2310763*qd5*sin(theta6))/3259964 + (63931*qd5)/13039856 - qd6/2)*sin(theta3)*(qd2 + qd3)*sin(theta2) + 13039856*(((16011145*qd5)/6519928 + qd5*cos(theta6)^2 - (2310763*qd6*sin(theta6))/1629982)*sin(theta5) + 2*qd4*sin(theta6)*cos(theta6) - (46480089*qd4)/3259964)*qd1)*cos(theta5) + 13039856*sin(theta3)*(((-qd5*sin(theta6) - (2310763*qd6)/1629982)*cos(theta6) + (46480089*qd5)/6519928)*sin(theta5) + qd4*(cos(theta6)^2 + 90090735/3259964))*(qd2 + qd3)*sin(theta2) + 13039856*(-2310763*(-9133/1320436 + sin(theta6))*qd4*sin(theta5)/814991 + (qd6*sin(theta6) - (2310763*qd5)/1629982)*cos(theta6) + (5043*qd5)/814991 + (510879*qd4)/1629982)*qd1)*cos(theta4)^2)/1000000000 + (((-13039856*sin(theta3)*((((2310763*qd5)/814991 + qd6*sin(theta6))*cos(theta6) - (10086*qd5)/814991)*(qd2 + qd3)*sin(theta4) + ((16011145*qd5)/6519928 + qd5*cos(theta6)^2 - (2310763*qd6*sin(theta6))/1629982)*qd4)*sin(theta2) + 13039856*(qd4*(16011145/6519928 + cos(theta6)^2)*sin(theta4) + 2310763*(cos(theta6) - 10086/2310763)*(qd2 + qd3)/814991)*qd1)*cos(theta5)^2 + ((((-13039856*((16011145*qd5)/6519928 + qd5*cos(theta6)^2 - (2310763*qd6*sin(theta6))/1629982)*(qd2 + qd3)*sin(theta4) + 13039856*(((2310763*qd5)/814991 + qd6*sin(theta6))*cos(theta6) - (10086*qd5)/814991)*qd4)*sin(theta5) - 26079712*(sin(theta6)*cos(theta6) - 46480089/6519928)*qd4*(qd2 + qd3)*sin(theta4) + 13039856*cos(theta6)^2*qd5*qd6 + (-9243052*qd2^2 - 18486104*qd2*qd3 - 9243052*qd3^2 + 9243052*qd4^2 - 9243052*qd5^2 + 9243052*qd6^2)*sin(theta6) + 63931*qd2^2 + 127862*qd2*qd3 + 63931*qd3^2 - 63931*qd4^2 - 2166000*qd4*qd5 + 63931*qd5^2 - 13045956*qd5*qd6)*sin(theta3) - 2052000*qd4*qd5)*sin(theta2) + 13039856*(-2310763*(cos(theta6) - 10086/2310763)*qd4*sin(theta4)/814991 + (16011145/6519928 + cos(theta6)^2)*(qd2 + qd3))*qd1*sin(theta5) + 26079712*qd1*(qd6*cos(theta6)^2 - (2310763*qd5*sin(theta6))/3259964 + (63931*qd5)/13039856 - qd6/2)*sin(theta4) + 399000*qd4*qd5)*cos(theta5) + (((36972208*(-9133/1320436 + sin(theta6))*qd4*(qd2 + qd3)*sin(theta4) - 6519928*sin(theta6)*(qd2^2 + 2*qd2*qd3 + qd3^2 - qd4^2 + qd5^2)*cos(theta6) + (-399000*qd2 - 399000*qd3)*qd1 + 46480089*qd2^2 + 92960178*qd2*qd3 + 46480089*qd3^2 - 46480089*qd4^2 + 46480089*qd5^2)*sin(theta5) - 13039856*((qd6*sin(theta6) - (2310763*qd5)/1629982)*cos(theta6) + (5043*qd5)/814991 + (510879*qd4)/1629982)*(qd2 + qd3)*sin(theta4) + 13039856*cos(theta6)^2*qd4*qd5 + 58876307*qd2^2 + 117752614*qd2*qd3 + 58876307*qd3^2 - 58876307*qd4^2 + 58705327*qd4*qd5)*sin(theta3) + 57348000*qd2^2 - 57348000*qd4^2)*sin(theta2) + 2052000*qd1*sin(theta5)*(qd2 + qd3)*sin(theta3) - 13039856*(((qd5*sin(theta6) + (2310763*qd6)/1629982)*cos(theta6) - (46480089*qd5)/6519928)*sin(theta4) - (135375*qd2)/814991 - (135375*qd3)/814991)*qd1*sin(theta5) + 13039856*qd4*qd1*(cos(theta6)^2 + 90090735/3259964)*sin(theta4) - 18486104*(qd2 + qd3)*qd1*cos(theta6) + (960136860*qd2 + 960136860*qd3)*qd1 + 11151000*qd4^2)*cos(theta4))/1000000000 - (814991*sin(theta2)*sin(theta3)*(2310763*(cos(theta6) - 10086/2310763)*(qd2 + qd3 - qd4)*(qd2 + qd3 + qd4)*sin(theta4)/1629982 + (16011145/6519928 + cos(theta6)^2)*qd4*(qd2 + qd3))*cos(theta5)^2)/62500000 + ((-6519928*(((16011145/6519928 + cos(theta6)^2)*(qd2 + qd3 - qd4)*(qd2 + qd3 + qd4)*sin(theta4) - 4621526*(cos(theta6) - 10086/2310763)*qd4*(qd2 + qd3)/814991)*sin(theta5) + 2*qd6*(-(2310763*qd4*cos(theta6)*sin(theta4))/1629982 + (cos(theta6)^2 + 1525/3259964)*(qd2 + qd3)))*sin(theta3)*sin(theta2) - 13039856*(2310763*(-9133/1320436 + sin(theta6))*(qd2 + qd3)*sin(theta4)/1629982 + (sin(theta6)*cos(theta6) - 46480089/6519928)*qd4)*qd1)*cos(theta5))/1000000000 + (((((13039856*cos(theta6)^2*qd4*qd6 - 1083000*qd2^2 - 2166000*qd2*qd3 - 1083000*qd3^2 + 1083000*qd4^2 + 6100*qd4*qd6 + 1083000*qd5^2)*sin(theta4) + 18486104*qd6*(qd2 + qd3)*cos(theta6) - 399000*qd1*qd5)*sin(theta5) + ((-13039856*sin(theta6)*qd5*qd6 + 9243052*qd2^2 + 18486104*qd2*qd3 + 9243052*qd3^2 - 9243052*qd4^2 + 9243052*qd6^2)*cos(theta6) + (-22302000*qd2 - 22302000*qd3)*qd1 - 480068430*(qd2 + qd3 + qd4)*(qd2 + qd3 - qd4))*sin(theta4) + 42223519*(qd2 + qd3 - (554059067*qd4)/42223519)*(qd2 + qd3))*sin(theta3) - 1026000*sin(theta4)*(qd2^2 - qd4^2 - qd5^2)*sin(theta5) - 253228718*qd2^2)*sin(theta2))/1000000000 + (14337*qd1*((19*qd5*sin(theta5))/1062 + sin(theta4)*(qd2 + qd3))*sin(theta3))/125000 + (((-13039856*qd1*sin(theta6)*(qd2 + qd3)*cos(theta6) + (92960178*qd2 + 92960178*qd3)*qd1 - 199500*qd4^2 - 199500*qd5^2)*sin(theta4) + 18486104*(-(9133*qd4)/1320436 + (270750*qd5)/2310763 + sin(theta6)*qd4)*qd1)*sin(theta5))/1000000000 - 814991*((-(58876307*qd2)/6519928 - (58876307*qd3)/6519928)*sin(theta4) + qd6*sin(theta6)*cos(theta6) + (11286963*qd2)/1629982 + (2389617*qd3)/6519928 + (510879*qd4)/3259964)*qd1/62500000;
v2 = (((-13039856*sin(theta2)*qd1^2*(cos(theta6)^2 + 16011145/6519928)*cos(theta2)*cos(theta3)^2 - 13039856*(qd1*cos(theta2)^2*sin(theta3) - qd1*sin(theta3)/2 + cos(theta2)*qd4)*qd1*(cos(theta6)^2 + 16011145/6519928)*cos(theta3) + 6519928*sin(theta2)*qd1^2*(cos(theta6)^2 + 16011145/6519928)*cos(theta2) + 13039856*qd4*qd1*sin(theta3)*cos(theta6)^2*sin(theta2) - 13039856*(qd6*sin(theta6) + (2310763*qd5)/814991)*(qd2 + qd3)*cos(theta6) + 32022290*qd1*qd4*sin(theta3)*sin(theta2) + 161376*qd5*(qd2 + qd3))*cos(theta5)^2 + (36972208*sin(theta5)*sin(theta2)*(cos(theta6) - 10086/2310763)*qd1^2*cos(theta2)*cos(theta3)^2 + 36972208*(qd1*sin(theta3)*sin(theta5)*(cos(theta6) - 10086/2310763)*cos(theta2)^2 + (qd4*(cos(theta6) - 10086/2310763)*sin(theta5) - (1629982*cos(theta6)^2*qd6)/2310763 + qd5*sin(theta6)/2 - (9133*qd5)/2640872 + (814991*qd6)/2310763)*cos(theta2) - qd1*sin(theta3)*sin(theta5)*(cos(theta6) - 10086/2310763)/2)*qd1*cos(theta3) - 18486104*sin(theta5)*sin(theta2)*(cos(theta6) - 10086/2310763)*qd1^2*cos(theta2) + (-13039856*qd5*(qd2 + qd3)*cos(theta6)^2 - 36972208*qd1*cos(theta6)*sin(theta2)*sin(theta3)*qd4 + 161376*qd1*qd4*sin(theta3)*sin(theta2) + 18486104*(qd6*sin(theta6) - (16011145*qd5)/9243052)*(qd2 + qd3))*sin(theta5) + 26079712*qd1*cos(theta6)^2*sin(theta2)*sin(theta3)*qd6 - 26079712*sin(theta6)*qd4*(qd2 + qd3)*cos(theta6) - 18486104*sin(theta2)*qd1*(qd5*sin(theta6) - (9133*qd5)/1320436 + (1629982*qd6)/2310763)*sin(theta3) + 185920356*qd4*(qd2 + qd3))*cos(theta5) - 13039856*sin(theta2)*qd1^2*(cos(theta6)^2 + 90090735/3259964)*cos(theta2)*cos(theta3)^2 - 13039856*(qd1*sin(theta3)*(cos(theta6)^2 + 90090735/3259964)*cos(theta2)^2 + (((-qd5*sin(theta6) - (2310763*qd6)/1629982)*cos(theta6) + (46480089*qd5)/6519928)*sin(theta5) + qd4*(cos(theta6)^2 + 90090735/3259964))*cos(theta2) - qd1*sin(theta3)*(cos(theta6)^2 + 90090735/3259964)/2)*qd1*cos(theta3) + 6519928*sin(theta2)*qd1^2*(cos(theta6)^2 + 90090735/3259964)*cos(theta2) + (-13039856*sin(theta2)*(qd5*sin(theta6) + (2310763*qd6)/1629982)*sin(theta3)*qd1*cos(theta6) + 92960178*qd1*sin(theta2)*sin(theta3)*qd5 + 36972208*qd4*(-9133/1320436 + sin(theta6))*(qd2 + qd3))*sin(theta5) + 13039856*qd4*qd1*sin(theta3)*cos(theta6)^2*sin(theta2) - 13039856*(qd6*sin(theta6) - (2310763*qd5)/1629982)*(qd2 + qd3)*cos(theta6) + 360362940*qd1*qd4*sin(theta3)*sin(theta2) - 4087032*(qd4 + (3362*qd5)/170293)*(qd2 + qd3))*cos(theta4)^2)/1000000000 + (((-73944416*(cos(theta6) - 10086/2310763)*(cos(theta2)^2 - 1/2)*qd1^2*cos(theta3)^2 + 73944416*qd1*(((((814991*qd6*sin(theta6))/4621526 + qd5/2)*cos(theta6) - (5043*qd5)/2310763)*sin(theta4) + qd1*sin(theta2)*sin(theta3)*(cos(theta6) - 10086/2310763))*cos(theta2) + sin(theta2)*(cos(theta6) - 10086/2310763)*qd4/2)*cos(theta3) + (36972208*qd1^2*cos(theta6) - 161376*qd1^2)*cos(theta2)^2 + 36972208*(cos(theta6) - 10086/2310763)*qd4*sin(theta3)*qd1*cos(theta2) + (-13039856*qd4*(qd2 + qd3)*cos(theta6)^2 - 13039856*sin(theta2)*sin(theta3)*(qd6*sin(theta6) + (2310763*qd5)/814991)*qd1*cos(theta6) + 161376*qd1*sin(theta2)*sin(theta3)*qd5 - 32022290*qd4*(qd2 + qd3))*sin(theta4) - 18486104*(cos(theta6) - 10086/2310763)*(qd1 + qd4)*(qd1 - qd4))*cos(theta5)^2 + (-26079712*(sin(theta5)*(cos(theta6)^2 + 16011145/6519928)*cos(theta2)^2 - sin(theta2)*(cos(theta6)*sin(theta6) - 46480089/6519928)*sin(theta4)*cos(theta2) - sin(theta5)*(cos(theta6)^2 + 16011145/6519928)/2)*qd1^2*cos(theta3)^2 + (26079712*sin(theta3)*(cos(theta6)*sin(theta6) - 46480089/6519928)*qd1^2*sin(theta4)*cos(theta2)^2 + 26079712*qd1*(((qd5*cos(theta6)^2/2 - (2310763*qd6*sin(theta6))/3259964 + (16011145*qd5)/13039856)*sin(theta5) + qd4*(cos(theta6)*sin(theta6) - 46480089/6519928))*sin(theta4) + qd1*sin(theta2)*sin(theta3)*sin(theta5)*(cos(theta6)^2 + 16011145/6519928))*cos(theta2) - 13039856*sin(theta3)*(cos(theta6)*sin(theta6) - 46480089/6519928)*qd1^2*sin(theta4) + 13039856*sin(theta2)*qd4*qd1*(cos(theta6)^2 + 16011145/6519928)*sin(theta5) + 18486104*qd1*cos(theta6)*sin(theta2)*qd6 - 2052000*qd5*(qd2 + qd3))*cos(theta3) + 13039856*sin(theta5)*qd1^2*(cos(theta6)^2 + 16011145/6519928)*cos(theta2)^2 - 13039856*(qd1*sin(theta2)*(cos(theta6)*sin(theta6) - 46480089/6519928)*sin(theta4) - (qd4*(cos(theta6)^2 + 16011145/6519928)*sin(theta5) + (2310763*qd6*cos(theta6))/1629982)*sin(theta3))*qd1*cos(theta2) + ((-13039856*qd1*cos(theta6)^2*sin(theta2)*sin(theta3)*qd5 + 36972208*qd4*(qd2 + qd3)*cos(theta6) + 18486104*(qd6*sin(theta6) - (16011145*qd5)/9243052)*sin(theta2)*qd1*sin(theta3) - 161376*qd4*(qd2 + qd3))*sin(theta5) - 26079712*qd6*(qd2 + qd3)*cos(theta6)^2 - 26079712*qd1*cos(theta6)*sin(theta2)*sin(theta3)*sin(theta6)*qd4 + 185920356*qd1*qd4*sin(theta3)*sin(theta2) + 18486104*(qd2 + qd3)*(qd5*sin(theta6) - (9133*qd5)/1320436 + (1629982*qd6)/2310763))*sin(theta4) - 6519928*(cos(theta6)^2 + 16011145/6519928)*(qd1 + qd4)*(qd1 - qd4)*sin(theta5) + 18486104*cos(theta6)*qd4*qd6)*cos(theta5) + 36972208*qd1^2*((cos(theta6) - (270750*sin(theta5))/2310763 - 240034215/4621526)*cos(theta2)^2 - sin(theta2)*(-510879/4621526 + (-9133/1320436 + sin(theta6))*sin(theta5))*sin(theta4)*cos(theta2) - cos(theta6)/2 + (135375*sin(theta5))/2310763 + 240034215/9243052)*cos(theta3)^2 + (-36972208*(-510879/4621526 + (-9133/1320436 + sin(theta6))*sin(theta5))*sin(theta3)*qd1^2*sin(theta4)*cos(theta2)^2 - 36972208*((qd4*(-9133/1320436 + sin(theta6))*sin(theta5) + (-(814991*qd6*sin(theta6))/2310763 + qd5/2)*cos(theta6) - (510879*qd4)/4621526 - (5043*qd5)/2310763)*sin(theta4) + ((-(270750*sin(theta2)*sin(theta3))/2310763 - (128250*sin(theta2))/2310763 + 7125/1320436)*sin(theta5) + sin(theta2)*sin(theta3)*(cos(theta6) - 240034215/4621526))*qd1)*qd1*cos(theta2) + 18486104*(-510879/4621526 + (-9133/1320436 + sin(theta6))*sin(theta5))*sin(theta3)*qd1^2*sin(theta4) + 13039856*sin(theta2)*(cos(theta6)^2*qd6 + (135375*qd4)/814991 + (1525*qd6)/3259964)*qd1*sin(theta5) - 18486104*qd4*(qd1*cos(theta6)*sin(theta2) - (240034215*qd1*sin(theta2))/4621526 + (14337000*qd2)/2310763 + (14337000*qd3)/2310763))*cos(theta3) + (2052000*qd1^2*(sin(theta3) + 19/18)*sin(theta5) - 18486104*qd1^2*cos(theta6) + 960136860*qd1^2)*cos(theta2)^2 + 18486104*(sin(theta2)*(-510879/4621526 + (-9133/1320436 + sin(theta6))*sin(theta5))*qd1*sin(theta4) + ((1629982*cos(theta6)^2*sin(theta3)*qd6)/2310763 + ((270750*qd4)/2310763 + (1525*qd6)/4621526)*sin(theta3) + (256500*qd4)/2310763)*sin(theta5) - qd4*sin(theta3)*(cos(theta6) - 240034215/4621526))*qd1*cos(theta2) + ((13039856*(qd5*sin(theta6) + (2310763*qd6)/1629982)*(qd2 + qd3)*cos(theta6) + 36972208*sin(theta2)*qd4*qd1*(-9133/1320436 + sin(theta6))*sin(theta3) - 92960178*qd5*(qd2 + qd3))*sin(theta5) - 13039856*qd4*(qd2 + qd3)*cos(theta6)^2 - 13039856*sin(theta2)*(qd6*sin(theta6) - (2310763*qd5)/1629982)*sin(theta3)*qd1*cos(theta6) - 4087032*(qd4 + (3362*qd5)/170293)*sin(theta2)*qd1*sin(theta3) - 360362940*qd4*(qd2 + qd3))*sin(theta4) + (13039856*cos(theta6)^2*qd4*qd6 + (199500*qd1^2*sin(theta2) - 1026000*qd1^2 + 1026000*qd4^2 + 1026000*qd5^2 + 2052000*qd3*(qd2 + qd3/2))*sin(theta3) - 1083000*qd1^2 + 1083000*qd4^2 + 6100*qd6*qd4 + 1083000*qd5^2)*sin(theta5) + (-13039856*sin(theta6)*qd5*qd6 + 9243052*qd1^2 - 9243052*qd4^2 + 9243052*qd6^2)*cos(theta6) - 480068430*qd1^2 + 480068430*qd4^2)*cos(theta4))/1000000000 + ((-13039856*sin(theta2)*qd1^2*(cos(theta6)^2 + 16011145/6519928)*cos(theta2)*cos(theta3)^2 - 13039856*qd1*(qd1*sin(theta3)*(cos(theta6)^2 + 16011145/6519928)*cos(theta2)^2 - sin(theta2)*(qd5*cos(theta6)^2 - (2310763*qd6*sin(theta6))/1629982 + (16011145*qd5)/6519928)*sin(theta4) - qd1*sin(theta3)*(cos(theta6)^2 + 16011145/6519928)/2)*cos(theta3) + 6519928*(2*(qd5*cos(theta6)^2 - (2310763*qd6*sin(theta6))/1629982 + (16011145*qd5)/6519928)*sin(theta3)*sin(theta4) + qd1*sin(theta2)*(cos(theta6)^2 + 16011145/6519928))*qd1*cos(theta2) + (13039856*cos(theta6)^2*qd4*qd5 - 18486104*sin(theta6)*qd4*qd6 + 32022290*qd4*qd5)*sin(theta4) + 13039856*((qd6*sin(theta6) + (2310763*qd5)/814991)*cos(theta6) - (10086*qd5)/814991)*(qd2 + qd3))*cos(theta5)^2)/1000000000 + ((36972208*(sin(theta4)*(-9133/1320436 + sin(theta6))*cos(theta2)^2 + sin(theta2)*(-270750/2310763 + (cos(theta6) - 10086/2310763)*sin(theta5))*cos(theta2) - sin(theta4)*(-9133/1320436 + sin(theta6))/2)*qd1^2*cos(theta3)^2 + (36972208*(sin(theta3)*(cos(theta6) - 10086/2310763)*sin(theta5) - (270750*sin(theta3))/2310763 - 128250/2310763)*qd1^2*cos(theta2)^2 - 36972208*qd1*(qd1*sin(theta2)*sin(theta3)*(-9133/1320436 + sin(theta6))*sin(theta4) - (814991*cos(theta6)^2*qd6)/2310763 + qd5*sin(theta6)/2 - (9133*qd5)/2640872 + (465927*qd6)/1320436)*cos(theta2) - 13039856*sin(theta2)*(((qd6*sin(theta6) + (2310763*qd5)/814991)*cos(theta6) - (10086*qd5)/814991)*sin(theta5) + (2310763*sin(theta6)*qd4)/1629982 - (63931*qd4)/6519928 - (135375*qd5)/814991)*qd1*sin(theta4) - 18486104*(cos(theta6) - 10086/2310763)*sin(theta3)*qd1^2*sin(theta5) + 2166000*qd1^2*sin(theta3) - 199500*qd1^2*sin(theta2) + 1026000*qd1^2 - 1026000*qd5^2 - 2052000*qd3*(qd2 + qd3/2))*cos(theta3) - 18486104*qd1^2*(-9133/1320436 + sin(theta6))*sin(theta4)*cos(theta2)^2 - 18486104*((1629982*((qd6*sin(theta6) + (2310763*qd5)/814991)*cos(theta6) - (10086*qd5)/814991)*sin(theta3)*sin(theta5)/2310763 + (sin(theta6)*qd4 - (9133*qd4)/1320436 - (270750*qd5)/2310763)*sin(theta3) - (256500*qd5)/2310763)*sin(theta4) + qd1*(sin(theta5)*sin(theta2)*(cos(theta6) - 10086/2310763) + (-(256500*sin(theta2))/2310763 + 7125/660218)*sin(theta3) - (270750*sin(theta2))/2310763))*qd1*cos(theta2) + (-13039856*((qd6*sin(theta6) + (2310763*qd5)/814991)*cos(theta6) - (10086*qd5)/814991)*qd4*sin(theta5) - 13039856*cos(theta6)^2*qd5*qd6 + 2052000*sin(theta3)*qd4*qd5 + (9243052*qd1^2 - 9243052*qd4^2 + 9243052*qd5^2 - 9243052*qd6^2)*sin(theta6) - 63931*qd1^2 + 63931*qd4^2 + 2166000*qd4*qd5 - 63931*qd5^2 + 13045956*qd5*qd6)*sin(theta4) + 13039856*(qd5*cos(theta6)^2 - (2310763*qd6*sin(theta6))/1629982 + (16011145*qd5)/6519928)*(qd2 + qd3)*sin(theta5) - 13039856*qd1*cos(theta6)^2*sin(theta2)*sin(theta3)*qd6 + 13039856*sin(theta6)*qd4*(qd2 + qd3)*cos(theta6) + 18486104*sin(theta2)*qd1*(qd5*sin(theta6) - (9133*qd5)/1320436 + (465927*qd6)/660218)*sin(theta3) - 92960178*qd4*(qd2 + qd3))*cos(theta5))/1000000000 + 814991*((2389617/6519928 + (-58876307/6519928 + (cos(theta6)*sin(theta6) - 46480089/6519928)*sin(theta5))*sin(theta4))*cos(theta2)^2 + sin(theta2)*(cos(theta6)^2 + 510474629/6519928)*cos(theta2) - 2389617/13039856 + (58876307/13039856 + (-cos(theta6)*sin(theta6)/2 + 46480089/13039856)*sin(theta5))*sin(theta4))*qd1^2*cos(theta3)^2/31250000 + (((26079712*qd1^2*cos(theta6)^2*sin(theta3) + 2041898516*qd1^2*sin(theta3) - 15048000*qd1^2)*cos(theta2)^2 - 26079712*(qd1*(sin(theta2)*sin(theta3)*(cos(theta6)*sin(theta6) - 46480089/6519928)*sin(theta5) - (58876307*sin(theta2)*sin(theta3))/6519928 - (3584250*sin(theta2))/814991 + 1393875/3259964)*sin(theta4) + qd5*(cos(theta6)*sin(theta6) - 46480089/6519928)*sin(theta5)/2 + (2389617*qd1*sin(theta2)*sin(theta3))/6519928 - qd4*cos(theta6)^2/2 + (193696127*qd4)/26079712)*qd1*cos(theta2) + (-13039856*(qd1*cos(theta6)*sin(theta2)*sin(theta6) - (46480089*qd1*sin(theta2))/6519928 - (128250*qd2)/814991 - (128250*qd3)/814991)*qd4*sin(theta5) - 13039856*sin(theta2)*qd1*(qd5*cos(theta6)^2 - (58876307*qd4)/6519928 + (58705327*qd5)/13039856))*sin(theta4) - 13039856*qd1^2*cos(theta6)^2*sin(theta3) - 1020949258*qd1^2*sin(theta3) - 1463000*qd1^2*sin(theta2) + 7524000*qd1^2 - 15048000*qd3*(qd2 + qd3/2))*cos(theta3))/1000000000 - 814991*(11286963/1629982 + ((cos(theta6)*sin(theta6) - 46480089/6519928)*sin(theta5) - (7168500*sin(theta3))/814991 - 58876307/6519928)*sin(theta4))*qd1^2*cos(theta2)^2/62500000 - (814991*qd1*((qd4*sin(theta3)*(cos(theta6)*sin(theta6) - 46480089/6519928)*sin(theta5) + cos(theta6)^2*sin(theta3)*qd5 + (-(58876307*qd4)/6519928 + (58705327*qd5)/13039856)*sin(theta3) - (7168500*qd4)/814991)*sin(theta4) + (sin(theta2)*cos(theta6)^2 + (-(940500*sin(theta2))/814991 + 182875/1629982)*sin(theta3) + (2497191253*sin(theta2))/13039856 - 21672000/814991)*qd1)*cos(theta2))/62500000 + ((6519928*(qd1^2 - qd4^2 + qd5^2)*(cos(theta6)*sin(theta6) - 46480089/6519928)*sin(theta5) - 13039856*cos(theta6)^2*qd4*qd5 + (11151000*qd1^2*sin(theta2) - 57348000*qd1^2 + 57348000*qd4^2 + 114696000*qd3*(qd2 + qd3/2))*sin(theta3) - 58876307*qd1^2 + 58876307*qd4^2 - 58705327*qd4*qd5)*sin(theta4))/1000000000 + ((13039856*qd1*cos(theta6)*sin(theta2)*sin(theta3)*sin(theta6)*qd5 + (-92960178*qd1*sin(theta2)*qd5 + 2052000*qd5*(qd2 + qd3))*sin(theta3) - 18486104*(sin(theta6)*qd4 - (9133*qd4)/1320436 - (270750*qd5)/2310763)*(qd2 + qd3))*sin(theta5))/1000000000 - (814991*qd4*qd1*sin(theta3)*cos(theta6)^2*sin(theta2))/62500000 - (2310763*qd5*(qd2 + qd3)*cos(theta6))/125000000 + (193696127*qd1*qd4*sin(theta3)*sin(theta2))/1000000000 + (11286963*qd1^2)/250000000 + 510879*(qd4 + (6724*qd5)/170293)*(qd2 + qd3)/250000000;
v3 = (((-13039856*(cos(theta6)^2 + 16011145/6519928)*sin(theta3)*qd1^2*cos(theta3)*cos(theta2)^2 - 13039856*(cos(theta6)^2 + 16011145/6519928)*qd1*(qd1*cos(theta3)^2*sin(theta2) - qd1*sin(theta2)/2 + cos(theta3)*qd4)*cos(theta2) + 6519928*(cos(theta6)^2 + 16011145/6519928)*sin(theta3)*qd1^2*cos(theta3) + 13039856*qd4*qd1*sin(theta3)*sin(theta2)*cos(theta6)^2 - 13039856*(qd6*sin(theta6) + (2310763*qd5)/814991)*(qd2 + qd3)*cos(theta6) + 32022290*qd4*qd1*sin(theta3)*sin(theta2) + 161376*qd5*(qd2 + qd3))*cos(theta5)^2 + (36972208*sin(theta5)*(cos(theta6) - 10086/2310763)*sin(theta3)*qd1^2*cos(theta3)*cos(theta2)^2 + 36972208*(qd1*sin(theta2)*sin(theta5)*(cos(theta6) - 10086/2310763)*cos(theta3)^2 + (-(1629982*cos(theta6)^2*qd6)/2310763 + cos(theta6)*sin(theta5)*qd4 - (10086*qd4*sin(theta5))/2310763 + qd5*sin(theta6)/2 - (9133*qd5)/2640872 + (814991*qd6)/2310763)*cos(theta3) - qd1*sin(theta2)*sin(theta5)*(cos(theta6) - 10086/2310763)/2)*qd1*cos(theta2) - 18486104*sin(theta5)*(cos(theta6) - 10086/2310763)*sin(theta3)*qd1^2*cos(theta3) + (-13039856*qd5*(qd2 + qd3)*sin(theta5) + 26079712*qd1*sin(theta2)*sin(theta3)*qd6)*cos(theta6)^2 - 36972208*qd4*(qd1*sin(theta2)*sin(theta3)*sin(theta5) + (1629982*sin(theta6)*(qd2 + qd3))/2310763)*cos(theta6) + (161376*qd4*qd1*sin(theta3)*sin(theta2) + 18486104*(qd6*sin(theta6) - (16011145*qd5)/9243052)*(qd2 + qd3))*sin(theta5) - 18486104*sin(theta2)*qd1*(qd5*sin(theta6) - (9133*qd5)/1320436 + (1629982*qd6)/2310763)*sin(theta3) + 185920356*qd4*(qd2 + qd3))*cos(theta5) - 13039856*(cos(theta6)^2 + 90090735/3259964)*sin(theta3)*qd1^2*cos(theta3)*cos(theta2)^2 - 13039856*qd1*(qd1*sin(theta2)*(cos(theta6)^2 + 90090735/3259964)*cos(theta3)^2 + (qd4*cos(theta6)^2 - sin(theta5)*(qd5*sin(theta6) + (2310763*qd6)/1629982)*cos(theta6) + (46480089*qd5*sin(theta5))/6519928 + (90090735*qd4)/3259964)*cos(theta3) - qd1*sin(theta2)*(cos(theta6)^2 + 90090735/3259964)/2)*cos(theta2) + 6519928*(cos(theta6)^2 + 90090735/3259964)*sin(theta3)*qd1^2*cos(theta3) + 13039856*qd4*qd1*sin(theta3)*sin(theta2)*cos(theta6)^2 + (-13039856*sin(theta2)*(qd5*sin(theta6) + (2310763*qd6)/1629982)*sin(theta3)*qd1*sin(theta5) - 13039856*(qd6*sin(theta6) - (2310763*qd5)/1629982)*(qd2 + qd3))*cos(theta6) + (92960178*qd1*sin(theta2)*sin(theta3)*qd5 + 36972208*qd4*(-9133/1320436 + sin(theta6))*(qd2 + qd3))*sin(theta5) + 360362940*qd4*qd1*sin(theta3)*sin(theta2) - 4087032*(qd4 + (3362*qd5)/170293)*(qd2 + qd3))*cos(theta4)^2)/1000000000 + (((-73944416*(cos(theta6) - 10086/2310763)*(cos(theta3)^2 - 1/2)*qd1^2*cos(theta2)^2 + 73944416*qd1*(((((814991*qd6*sin(theta6))/4621526 + qd5/2)*cos(theta6) - (5043*qd5)/2310763)*sin(theta4) + qd1*sin(theta2)*sin(theta3)*(cos(theta6) - 10086/2310763))*cos(theta3) + ((cos(theta6) - 10086/2310763)*qd4*sin(theta3))/2)*cos(theta2) + (36972208*qd1^2*cos(theta6) - 161376*qd1^2)*cos(theta3)^2 + 36972208*sin(theta2)*(cos(theta6) - 10086/2310763)*qd4*qd1*cos(theta3) + (-13039856*qd4*(qd2 + qd3)*cos(theta6)^2 - 13039856*sin(theta2)*sin(theta3)*(qd6*sin(theta6) + (2310763*qd5)/814991)*qd1*cos(theta6) + 161376*qd1*sin(theta2)*sin(theta3)*qd5 - 32022290*qd4*(qd2 + qd3))*sin(theta4) - 18486104*(cos(theta6) - 10086/2310763)*(qd1 + qd4)*(qd1 - qd4))*cos(theta5)^2 + (-26079712*(sin(theta5)*(cos(theta6)^2 + 16011145/6519928)*cos(theta3)^2 - sin(theta3)*(cos(theta6)*sin(theta6) - 46480089/6519928)*sin(theta4)*cos(theta3) - sin(theta5)*(cos(theta6)^2 + 16011145/6519928)/2)*qd1^2*cos(theta2)^2 + 26079712*(qd1*sin(theta2)*sin(theta4)*(cos(theta6)*sin(theta6) - 46480089/6519928)*cos(theta3)^2 + ((qd5*sin(theta5)*cos(theta6)^2/2 + qd4*sin(theta6)*cos(theta6) + (-(2310763*qd6*sin(theta6))/3259964 + (16011145*qd5)/13039856)*sin(theta5) - (46480089*qd4)/6519928)*sin(theta4) + qd1*sin(theta2)*sin(theta3)*sin(theta5)*(cos(theta6)^2 + 16011145/6519928))*cos(theta3) - qd1*sin(theta2)*sin(theta4)*(cos(theta6)*sin(theta6) - 46480089/6519928)/2 + ((cos(theta6)^2*sin(theta5)*qd4 + (2310763*qd6*cos(theta6))/1629982 + (16011145*qd4*sin(theta5))/6519928)*sin(theta3))/2)*qd1*cos(theta2) + 13039856*sin(theta5)*(cos(theta6)^2 + 16011145/6519928)*qd1^2*cos(theta3)^2 - 13039856*(qd1*sin(theta3)*(cos(theta6)*sin(theta6) - 46480089/6519928)*sin(theta4) - sin(theta2)*(cos(theta6)^2*sin(theta5)*qd4 + (2310763*qd6*cos(theta6))/1629982 + (16011145*qd4*sin(theta5))/6519928))*qd1*cos(theta3) + ((-13039856*qd1*qd5*sin(theta3)*sin(theta2)*sin(theta5) - 26079712*qd6*(qd2 + qd3))*cos(theta6)^2 - 26079712*qd4*((-(2310763*qd2)/1629982 - (2310763*qd3)/1629982)*sin(theta5) + qd1*sin(theta2)*sin(theta3)*sin(theta6))*cos(theta6) + (18486104*(qd6*sin(theta6) - (16011145*qd5)/9243052)*sin(theta2)*qd1*sin(theta3) - 161376*qd4*(qd2 + qd3))*sin(theta5) + 185920356*qd4*qd1*sin(theta3)*sin(theta2) + 18486104*(qd2 + qd3)*(qd5*sin(theta6) - (9133*qd5)/1320436 + (1629982*qd6)/2310763))*sin(theta4) - 6519928*sin(theta5)*(qd1 - qd4)*(qd1 + qd4)*cos(theta6)^2 + 18486104*cos(theta6)*qd4*qd6 - 16011145*sin(theta5)*(qd1 - qd4)*(qd1 + qd4))*cos(theta5) + 36972208*((cos(theta6) - (270750*sin(theta5))/2310763 - 240034215/4621526)*cos(theta3)^2 - (-510879/4621526 + (-9133/1320436 + sin(theta6))*sin(theta5))*sin(theta3)*sin(theta4)*cos(theta3) - cos(theta6)/2 + 240034215/9243052 + ((64125*sin(theta3))/2310763 + 135375/2310763)*sin(theta5))*qd1^2*cos(theta2)^2 - 36972208*qd1*(sin(theta2)*(-510879/4621526 + (-9133/1320436 + sin(theta6))*sin(theta5))*qd1*sin(theta4)*cos(theta3)^2 + (((-(814991*qd6*sin(theta6))/2310763 + qd5/2)*cos(theta6) + qd4*(-9133/1320436 + sin(theta6))*sin(theta5) - (510879*qd4)/4621526 - (5043*qd5)/2310763)*sin(theta4) + (cos(theta6)*sin(theta2)*sin(theta3) + (-(270750*sin(theta2)*sin(theta3))/2310763 - (64125*sin(theta2))/2310763 + 7125/1320436)*sin(theta5) - (240034215*sin(theta2)*sin(theta3))/4621526)*qd1)*cos(theta3) - sin(theta2)*(-510879/4621526 + (-9133/1320436 + sin(theta6))*sin(theta5))*qd1*sin(theta4)/2 - 814991*(cos(theta6)^2*sin(theta5)*qd6 - (2310763*cos(theta6)*qd4)/1629982 + ((135375*qd4)/814991 + (1525*qd6)/3259964)*sin(theta5) + (240034215*qd4)/3259964)*sin(theta3)/2310763)*cos(theta2) + (-18486104*qd1^2*cos(theta6) + 2166000*qd1^2*sin(theta5) + 960136860*qd1^2)*cos(theta3)^2 + 18486104*((-510879/4621526 + (-9133/1320436 + sin(theta6))*sin(theta5))*sin(theta3)*qd1*sin(theta4) + (1629982*sin(theta2)*(cos(theta6)^2*sin(theta5)*qd6 - (2310763*cos(theta6)*qd4)/1629982 + ((135375*qd4)/814991 + (1525*qd6)/3259964)*sin(theta5) + (240034215*qd4)/3259964))/2310763)*qd1*cos(theta3) + (-13039856*qd4*(qd2 + qd3)*cos(theta6)^2 + (13039856*(qd5*sin(theta6) + (2310763*qd6)/1629982)*(qd2 + qd3)*sin(theta5) - 13039856*sin(theta2)*(qd6*sin(theta6) - (2310763*qd5)/1629982)*sin(theta3)*qd1)*cos(theta6) + (36972208*sin(theta2)*qd4*qd1*(-9133/1320436 + sin(theta6))*sin(theta3) - 92960178*qd5*(qd2 + qd3))*sin(theta5) - 4087032*sin(theta2)*(qd4 + (3362*qd5)/170293)*qd1*sin(theta3) - 360362940*qd4*(qd2 + qd3))*sin(theta4) + 13039856*cos(theta6)^2*sin(theta5)*qd4*qd6 + (-13039856*sin(theta6)*qd5*qd6 + 9243052*qd1^2 - 9243052*qd4^2 + 9243052*qd6^2)*cos(theta6) + ((199500*qd1^2*sin(theta2) - 1026000*qd1^2 - 1026000*qd2^2)*sin(theta3) - 1083000*qd1^2 + 1083000*qd4^2 + 6100*qd4*qd6 + 1083000*qd5^2)*sin(theta5) - 480068430*qd1^2 + 480068430*qd4^2)*cos(theta4))/1000000000 + ((-13039856*(cos(theta6)^2 + 16011145/6519928)*sin(theta3)*qd1^2*cos(theta3)*cos(theta2)^2 - 13039856*(qd1*sin(theta2)*(cos(theta6)^2 + 16011145/6519928)*cos(theta3)^2 - (qd5*cos(theta6)^2 - (2310763*qd6*sin(theta6))/1629982 + (16011145*qd5)/6519928)*sin(theta3)*sin(theta4) - qd1*sin(theta2)*(cos(theta6)^2 + 16011145/6519928)/2)*qd1*cos(theta2) + 6519928*(2*sin(theta2)*(qd5*cos(theta6)^2 - (2310763*qd6*sin(theta6))/1629982 + (16011145*qd5)/6519928)*sin(theta4) + qd1*sin(theta3)*(cos(theta6)^2 + 16011145/6519928))*qd1*cos(theta3) + (13039856*cos(theta6)^2*qd4*qd5 - 18486104*sin(theta6)*qd4*qd6 + 32022290*qd4*qd5)*sin(theta4) + 13039856*((qd6*sin(theta6) + (2310763*qd5)/814991)*cos(theta6) - (10086*qd5)/814991)*(qd2 + qd3))*cos(theta5)^2)/1000000000 + ((36972208*qd1^2*(sin(theta4)*(-9133/1320436 + sin(theta6))*cos(theta3)^2 + (cos(theta6)*sin(theta3)*sin(theta5) - (10086*sin(theta5)*sin(theta3))/2310763 - (270750*sin(theta3))/2310763 - 64125/2310763)*cos(theta3) - sin(theta4)*(-9133/1320436 + sin(theta6))/2)*cos(theta2)^2 + 36972208*(qd1*sin(theta2)*(sin(theta5)*cos(theta6) - (10086*sin(theta5))/2310763 - 270750/2310763)*cos(theta3)^2 + (-sin(theta2)*sin(theta3)*qd1*(-9133/1320436 + sin(theta6))*sin(theta4) + (814991*cos(theta6)^2*qd6)/2310763 - qd5*sin(theta6)/2 + (9133*qd5)/2640872 - (465927*qd6)/1320436)*cos(theta3) - (814991*sin(theta3)*(sin(theta5)*(qd6*sin(theta6) + (2310763*qd5)/814991)*cos(theta6) - (10086*qd5*sin(theta5))/814991 + (2310763*sin(theta6)*qd4)/1629982 - (63931*qd4)/6519928 - (135375*qd5)/814991)*sin(theta4))/2310763 - ((sin(theta5)*sin(theta2)*cos(theta6) - (10086*sin(theta5)*sin(theta2))/2310763 + (-(128250*sin(theta2))/2310763 + 7125/660218)*sin(theta3) - (270750*sin(theta2))/2310763)*qd1)/2)*qd1*cos(theta2) - 18486104*qd1^2*(-9133/1320436 + sin(theta6))*sin(theta4)*cos(theta3)^2 + (-13039856*sin(theta2)*qd1*(sin(theta5)*(qd6*sin(theta6) + (2310763*qd5)/814991)*cos(theta6) - (10086*qd5*sin(theta5))/814991 + (2310763*sin(theta6)*qd4)/1629982 - (63931*qd4)/6519928 - (135375*qd5)/814991)*sin(theta4) - 18486104*qd1^2*cos(theta6)*sin(theta3)*sin(theta5) + 80688*qd1^2*sin(theta3)*sin(theta5) - 199500*qd1^2*sin(theta2) + 2166000*qd1^2*sin(theta3) + 1026000*qd1^2 + 1026000*qd2^2)*cos(theta3) + (-13039856*cos(theta6)^2*qd5*qd6 - 13039856*sin(theta5)*qd4*(qd6*sin(theta6) + (2310763*qd5)/814991)*cos(theta6) + 161376*sin(theta5)*qd4*qd5 + (9243052*qd1^2 - 9243052*qd4^2 + 9243052*qd5^2 - 9243052*qd6^2)*sin(theta6) - 63931*qd1^2 + 63931*qd4^2 + 2166000*qd4*qd5 - 63931*qd5^2 + 13045956*qd5*qd6)*sin(theta4) + (13039856*qd5*(qd2 + qd3)*sin(theta5) - 13039856*qd1*sin(theta2)*sin(theta3)*qd6)*cos(theta6)^2 + 13039856*sin(theta6)*qd4*(qd2 + qd3)*cos(theta6) - 18486104*(qd6*sin(theta6) - (16011145*qd5)/9243052)*(qd2 + qd3)*sin(theta5) + 18486104*sin(theta2)*qd1*(qd5*sin(theta6) - (9133*qd5)/1320436 + (465927*qd6)/660218)*sin(theta3) - 92960178*qd4*(qd2 + qd3))*cos(theta5))/1000000000 + 814991*((2389617/6519928 + (sin(theta5)*sin(theta6)*cos(theta6) - (46480089*sin(theta5))/6519928 - 58876307/6519928)*sin(theta4))*cos(theta3)^2 + (sin(theta3)*cos(theta6)^2 + (510474629*sin(theta3))/6519928 - 235125/814991)*cos(theta3) - 2389617/13039856 + (-sin(theta5)*sin(theta6)*cos(theta6)/2 + (1792125*sin(theta3))/814991 + (46480089*sin(theta5))/13039856 + 58876307/13039856)*sin(theta4))*qd1^2*cos(theta2)^2/31250000 + 814991*(qd1*sin(theta2)*(cos(theta6)^2 + 510474629/6519928)*cos(theta3)^2 + (-qd1*(sin(theta3)*sin(theta2)*sin(theta5)*sin(theta6)*cos(theta6) - (46480089*sin(theta3)*sin(theta2)*sin(theta5))/6519928 - (58876307*sin(theta2)*sin(theta3))/6519928 - (1792125*sin(theta2))/814991 + 1393875/3259964)*sin(theta4) - cos(theta6)*sin(theta5)*sin(theta6)*qd5/2 - (2389617*qd1*sin(theta2)*sin(theta3))/6519928 + qd4*cos(theta6)^2/2 + (46480089*qd5*sin(theta5))/13039856 - (193696127*qd4)/26079712)*cos(theta3) - sin(theta3)*(qd4*sin(theta6)*sin(theta5)*cos(theta6) + qd5*cos(theta6)^2 - (46480089*qd4*sin(theta5))/6519928 - (58876307*qd4)/6519928 + (58705327*qd5)/13039856)*sin(theta4)/2 - ((cos(theta6)^2*sin(theta2) + (-(470250*sin(theta2))/814991 + 182875/1629982)*sin(theta3) + (510474629*sin(theta2))/6519928)*qd1)/2)*qd1*cos(theta2)/31250000 - 814991*(2389617/6519928 + (sin(theta5)*sin(theta6)*cos(theta6) - (46480089*sin(theta5))/6519928 - 58876307/6519928)*sin(theta4))*qd1^2*cos(theta3)^2/62500000 + ((-13039856*sin(theta2)*qd1*(qd4*sin(theta6)*sin(theta5)*cos(theta6) + qd5*cos(theta6)^2 - (46480089*qd4*sin(theta5))/6519928 - (58876307*qd4)/6519928 + (58705327*qd5)/13039856)*sin(theta4) - 13039856*qd1^2*cos(theta6)^2*sin(theta3) - 1463000*qd1^2*sin(theta2) - 1020949258*qd1^2*sin(theta3) + 7524000*qd1^2 + 7524000*qd2^2)*cos(theta3))/1000000000 + ((-13039856*cos(theta6)^2*qd4*qd5 + 6519928*sin(theta5)*sin(theta6)*(qd1^2 - qd4^2 + qd5^2)*cos(theta6) + (-46480089*qd1^2 + 46480089*qd4^2 - 46480089*qd5^2)*sin(theta5) + (11151000*qd1^2*sin(theta2) - 57348000*qd1^2 - 57348000*qd2^2)*sin(theta3) - 58876307*qd1^2 + 58876307*qd4^2 - 58705327*qd4*qd5)*sin(theta4))/1000000000 - (814991*qd4*qd1*sin(theta3)*sin(theta2)*cos(theta6)^2)/62500000 + (814991*qd5*(qd1*sin(theta2)*sin(theta3)*sin(theta5)*sin(theta6) - (2310763*qd2)/1629982 - (2310763*qd3)/1629982)*cos(theta6))/62500000 + ((-92960178*qd1*sin(theta2)*sin(theta3)*qd5 - 18486104*(sin(theta6)*qd4 - (9133*qd4)/1320436 - (270750*qd5)/2310763)*(qd2 + qd3))*sin(theta5))/1000000000 + (193696127*qd4*qd1*sin(theta3)*sin(theta2))/1000000000 + (2389617*qd1^2)/1000000000 + 510879*(qd4 + (6724*qd5)/170293)*(qd2 + qd3)/250000000;
v4 = ((13039856*(cos(theta6)^2 + 16011145/6519928)*(cos(theta2)*cos(theta3) - sin(theta2)*sin(theta3))*qd1*(qd2 + qd3)*cos(theta5)^2 + (-26079712*(cos(theta3)^2 - 1/2)*(cos(theta6)*sin(theta6) - 46480089/6519928)*qd1^2*cos(theta2)^2 + 26079712*qd1*(-2310763*(cos(theta6) - 10086/2310763)*(qd2 + qd3)*sin(theta5)/1629982 + qd1*sin(theta2)*sin(theta3)*(cos(theta6)*sin(theta6) - 46480089/6519928))*cos(theta3)*cos(theta2) + (13039856*qd1^2*cos(theta6)*sin(theta6) - 92960178*qd1^2)*cos(theta3)^2 + 36972208*sin(theta2)*sin(theta3)*qd1*(cos(theta6) - 10086/2310763)*(qd2 + qd3)*sin(theta5) - 13039856*(qd1 + qd2 + qd3)*(qd1 - qd2 - qd3)*(cos(theta6)*sin(theta6) - 46480089/6519928))*cos(theta5) + 36972208*(-510879/4621526 + (-9133/1320436 + sin(theta6))*sin(theta5))*(cos(theta3)^2 - 1/2)*qd1^2*cos(theta2)^2 - 36972208*qd1*(qd1*sin(theta2)*sin(theta3)*(-9133/1320436 + sin(theta6))*sin(theta5) + (-(814991*qd2)/2310763 - (814991*qd3)/2310763)*cos(theta6)^2 - (510879*qd1*sin(theta2)*sin(theta3))/4621526 - (12870105*qd2)/1320436 - (12870105*qd3)/1320436)*cos(theta3)*cos(theta2) + ((-18486104*qd1^2*sin(theta6) + 127862*qd1^2)*sin(theta5) + 2043516*qd1^2)*cos(theta3)^2 + 18486104*(qd1 + qd2 + qd3)*(qd1 - qd2 - qd3)*(-9133/1320436 + sin(theta6))*sin(theta5) - 13039856*qd1*sin(theta2)*sin(theta3)*(qd2 + qd3)*cos(theta6)^2 - 360362940*qd1*sin(theta2)*sin(theta3)*(qd2 + qd3) - 2043516*(qd1 + qd2 + qd3)*(qd1 - qd2 - qd3))*cos(theta4)^2)/1000000000 + (((-13039856*(cos(theta6)^2 + 16011145/6519928)*(cos(theta3)^2 - 1/2)*qd1^2*sin(theta4)*cos(theta2)^2 + 13039856*qd1*((qd1*sin(theta2)*sin(theta3)*(cos(theta6)^2 + 16011145/6519928)*sin(theta4) + qd5*cos(theta6)^2 - (2310763*qd6*sin(theta6))/1629982 + (16011145*qd5)/6519928)*cos(theta3) - (2310763*sin(theta3)*(cos(theta6) - 10086/2310763)*(qd2 + qd3))/814991)*cos(theta2) + 6519928*(cos(theta6)^2 + 16011145/6519928)*qd1^2*sin(theta4)*cos(theta3)^2 - 36972208*sin(theta2)*qd1*(cos(theta6) - 10086/2310763)*(qd2 + qd3)*cos(theta3) - 6519928*(qd1 + qd2 + qd3)*(cos(theta6)^2 + 16011145/6519928)*(qd1 - qd2 - qd3)*sin(theta4) - 13039856*sin(theta2)*(qd5*cos(theta6)^2 - (2310763*qd6*sin(theta6))/1629982 + (16011145*qd5)/6519928)*sin(theta3)*qd1)*cos(theta5)^2 + (36972208*qd1^2*(sin(theta4)*sin(theta5)*(cos(theta6) - 10086/2310763)*cos(theta3)^2 + sin(theta3)*(-9133/1320436 + sin(theta6))*cos(theta3)/2 - sin(theta4)*sin(theta5)*(cos(theta6) - 10086/2310763)/2)*cos(theta2)^2 + 18486104*qd1*(qd1*sin(theta2)*(-9133/1320436 + sin(theta6))*cos(theta3)^2 + ((-2*sin(theta2)*sin(theta3)*qd1*(cos(theta6) - 10086/2310763)*sin(theta4) + (-(1629982*qd6*sin(theta6))/2310763 - 2*qd5)*cos(theta6) + (20172*qd5)/2310763)*sin(theta5) - 3259964*(cos(theta6)*sin(theta6) - 46480089/6519928)*sin(theta4)*(qd2 + qd3)/2310763)*cos(theta3) - 1629982*(cos(theta6)^2 + 16011145/6519928)*sin(theta3)*(qd2 + qd3)*sin(theta5)/2310763 - qd1*sin(theta2)*(-9133/1320436 + sin(theta6))/2)*cos(theta2) - 18486104*sin(theta5)*qd1^2*sin(theta4)*(cos(theta6) - 10086/2310763)*cos(theta3)^2 - 9243052*qd1*((3259964*sin(theta2)*(cos(theta6)^2 + 16011145/6519928)*(qd2 + qd3)*sin(theta5))/2310763 + qd1*sin(theta3)*(-9133/1320436 + sin(theta6)))*cos(theta3) + (18486104*(qd1 + qd2 + qd3)*(qd1 - qd2 - qd3)*(cos(theta6) - 10086/2310763)*sin(theta4) + 13039856*sin(theta2)*sin(theta3)*qd1*((qd6*sin(theta6) + (2310763*qd5)/814991)*cos(theta6) - (10086*qd5)/814991))*sin(theta5) + 26079712*(cos(theta6)*sin(theta6) - 46480089/6519928)*(qd1*sin(theta2)*sin(theta3)*sin(theta4) + qd5/2)*(qd2 + qd3))*cos(theta5) - 13039856*(sin(theta4)*(cos(theta6)^2 + 90090735/3259964)*cos(theta3)^2 + ((-cos(theta6)*sin(theta3)*sin(theta6) + (46480089*sin(theta3))/6519928)*sin(theta5) + (58876307*sin(theta3))/6519928 + 3584250/814991)*cos(theta3) + sin(theta4)*(-cos(theta6)^2/2 - 90090735/6519928))*qd1^2*cos(theta2)^2 + 13039856*(sin(theta2)*(-58876307/6519928 + (cos(theta6)*sin(theta6) - 46480089/6519928)*sin(theta5))*qd1*cos(theta3)^2 + ((2310763*sin(theta4)*(-9133/1320436 + sin(theta6))*(qd2 + qd3)*sin(theta5))/814991 + (qd1*cos(theta6)^2*sin(theta2)*sin(theta3) - (510879*qd2)/1629982 - (510879*qd3)/1629982 + (90090735*qd1*sin(theta2)*sin(theta3))/3259964)*sin(theta4) + (2310763*qd6*sin(theta6))/1629982 + (26683037*qd5)/13039856)*cos(theta3) + (-qd1*cos(theta6)*sin(theta2)*sin(theta6)/2 + (46480089*qd1*sin(theta2))/13039856 + (-(135375*qd2)/814991 - (135375*qd3)/814991)*sin(theta3) - (128250*qd2)/814991)*sin(theta5) + (2310763*sin(theta3)*(qd2 + qd3)*cos(theta6))/1629982 + 3584250*(58876307/57348000 + sin(theta3))*qd1*sin(theta2)/814991 - 1393875*(qd1 + (16002281*qd2)/185850 + (16002281*qd3)/185850)*sin(theta3)/1629982)*qd1*cos(theta2) + 6519928*(cos(theta6)^2 + 90090735/3259964)*qd1^2*sin(theta4)*cos(theta3)^2 + ((-6519928*qd1^2*cos(theta6)*sin(theta3)*sin(theta6) - 2166000*qd1*(qd2 + qd3)*sin(theta2) + 46480089*qd1^2*sin(theta3))*sin(theta5) + 18486104*qd1*(qd2 + qd3)*sin(theta2)*cos(theta6) - 11151000*(qd1 + (16002281*qd2)/185850 + (16002281*qd3)/185850)*qd1*sin(theta2) + 58876307*qd1^2*sin(theta3) + 57348000*qd1^2 + 57348000*qd2^2)*cos(theta3) - 36972208*(sin(theta2)*sin(theta3)*qd1*(-9133/1320436 + sin(theta6))*sin(theta4) - (814991*cos(theta6)^2*qd6)/2310763 + qd5*sin(theta6)/2 - (9133*qd5)/2640872 + (465927*qd6)/1320436)*(qd2 + qd3)*sin(theta5) + (-6519928*(qd1 + qd2 + qd3)*(qd1 - qd2 - qd3)*cos(theta6)^2 + 4087032*qd1*sin(theta2)*sin(theta3)*(qd2 + qd3) - 180181470*(qd1 + qd2 + qd3)*(qd1 - qd2 - qd3))*sin(theta4) - 18486104*sin(theta2)*(qd6*sin(theta6) + (26683037*qd5)/18486104)*sin(theta3)*qd1)*cos(theta4))/1000000000 + ((36972208*sin(theta3)*qd1^2*sin(theta4)*cos(theta3)*(cos(theta6) - 10086/2310763)*cos(theta2)^2 + 36972208*qd1*(qd1*sin(theta2)*sin(theta4)*(cos(theta6) - 10086/2310763)*cos(theta3)^2 - qd1*sin(theta2)*sin(theta4)*(cos(theta6) - 10086/2310763)/2 - (814991*sin(theta3)*((qd6*sin(theta6) + (2310763*qd5)/814991)*cos(theta6) - (10086*qd5)/814991))/2310763)*cos(theta2) - 18486104*(qd1*sin(theta3)*(cos(theta6) - 10086/2310763)*sin(theta4) + (1629982*sin(theta2)*((qd6*sin(theta6) + (2310763*qd5)/814991)*cos(theta6) - (10086*qd5)/814991))/2310763)*qd1*cos(theta3) + 13039856*(qd5*cos(theta6)^2 - (2310763*qd6*sin(theta6))/1629982 + (16011145*qd5)/6519928)*(qd2 + qd3)*sin(theta4) - 13039856*qd4*((qd6*sin(theta6) + (2310763*qd5)/814991)*cos(theta6) - (10086*qd5)/814991))*cos(theta5)^2)/1000000000 + ((13039856*((cos(theta6)*sin(theta6) - 46480089/6519928)*cos(theta3)^2 + sin(theta3)*sin(theta4)*sin(theta5)*(cos(theta6)^2 + 16011145/6519928)*cos(theta3) - cos(theta6)*sin(theta6)/2 + 46480089/13039856)*qd1^2*cos(theta2)^2 + 13039856*(qd1*sin(theta2)*sin(theta4)*sin(theta5)*(cos(theta6)^2 + 16011145/6519928)*cos(theta3)^2 - (qd1*sin(theta2)*sin(theta3) + qd5*sin(theta4))*(cos(theta6)*sin(theta6) - 46480089/6519928)*cos(theta3) + (-sin(theta2)*(cos(theta6)^2 + 16011145/6519928)*qd1*sin(theta4)/2 - (qd5*cos(theta6)^2 - (2310763*qd6*sin(theta6))/1629982 + (16011145*qd5)/6519928)*sin(theta3))*sin(theta5) + (2310763*sin(theta3)*sin(theta4)*(-9133/1320436 + sin(theta6))*(qd2 + qd3))/1629982)*qd1*cos(theta2) + (-6519928*qd1^2*cos(theta6)*sin(theta6) + 46480089*qd1^2)*cos(theta3)^2 - 6519928*qd1*((qd1*sin(theta3)*(cos(theta6)^2 + 16011145/6519928)*sin(theta4) + 2*sin(theta2)*(qd5*cos(theta6)^2 - (2310763*qd6*sin(theta6))/1629982 + (16011145*qd5)/6519928))*sin(theta5) - (2310763*sin(theta2)*sin(theta4)*(-9133/1320436 + sin(theta6))*(qd2 + qd3))/814991)*cos(theta3) + (-13039856*(qd2 + qd3)*((qd6*sin(theta6) + (2310763*qd5)/814991)*cos(theta6) - (10086*qd5)/814991)*sin(theta4) - 13039856*cos(theta6)^2*qd4*qd5 + 18486104*sin(theta6)*qd4*qd6 - 32022290*qd4*qd5)*sin(theta5) + 6519928*(2*qd1*sin(theta2)*sin(theta3)*sin(theta4)*qd5 + qd1^2 - (qd2 + qd3 + qd5)*(qd2 + qd3 - qd5))*(cos(theta6)*sin(theta6) - 46480089/6519928))*cos(theta5))/1000000000 - (2310763*qd1^2*((-510879/4621526 + (-9133/1320436 + sin(theta6))*sin(theta5))*cos(theta3)^2 + sin(theta4)*((-(270750*sin(theta3))/2310763 - 128250/2310763)*sin(theta5) + sin(theta3)*(cos(theta6) - 240034215/4621526))*cos(theta3) + 510879/9243052 + (-sin(theta6)/2 + 9133/2640872)*sin(theta5))*cos(theta2)^2)/125000000 - 2310763*(qd1*sin(theta2)*sin(theta4)*(cos(theta6) - (270750*sin(theta5))/2310763 - 240034215/4621526)*cos(theta3)^2 + ((((1629982*cos(theta6)^2*qd6)/2310763 - qd5*sin(theta6) + (9133*qd5)/1320436 - (465927*qd6)/660218)*sin(theta4) - qd1*sin(theta2)*sin(theta3)*(-9133/1320436 + sin(theta6)))*sin(theta5) + ((1629982*qd2)/2310763 + (1629982*qd3)/2310763)*cos(theta6)^2 + (510879*qd1*sin(theta2)*sin(theta3))/4621526 - (193696127*qd2)/18486104 - (193696127*qd3)/18486104)*cos(theta3) + 128250*(-(814991*sin(theta3)*sin(theta6)*(qd2 + qd3)*cos(theta6))/64125 + qd1*(sin(theta3) + 19/18)*sin(theta2) - 7*(qd1 - (15493363*qd2)/33250 - (15493363*qd3)/33250)*sin(theta3)/36)*sin(theta4)*sin(theta5)/2310763 + (-qd1*cos(theta6)*sin(theta2)/2 + (240034215*qd1*sin(theta2))/9243052 + ((8410901*qd2)/1320436 + (8410901*qd3)/1320436)*sin(theta3) + (14337000*qd2)/2310763)*sin(theta4) - 1629982*((qd6*sin(theta6) + (2310763*qd5)/1629982)*cos(theta6) - (5043*qd5)/814991)*sin(theta3)/2310763)*qd1*cos(theta2)/125000000 + (((9243052*qd1^2*sin(theta6) - 63931*qd1^2)*sin(theta5) - 1021758*qd1^2)*cos(theta3)^2)/1000000000 + ((199500*sin(theta4)*((3259964*qd1*sin(theta2)*sin(theta6)*(qd2 + qd3)*cos(theta6))/49875 + qd1*(qd1 - (15493363*qd2)/33250 - (15493363*qd3)/33250)*sin(theta2) - (38*qd1^2*sin(theta3))/7 - (36*qd1^2)/7 - (36*qd2^2)/7)*sin(theta5) + 9243052*qd1*((qd1*cos(theta6)*sin(theta3) + (-(8410901*qd2)/660218 - (8410901*qd3)/660218)*sin(theta2) - (240034215*qd1*sin(theta3))/4621526)*sin(theta4) + (3259964*sin(theta2)*((qd6*sin(theta6) + (2310763*qd5)/1629982)*cos(theta6) - (5043*qd5)/814991))/2310763))*cos(theta3))/1000000000 + ((13039856*sin(theta2)*(cos(theta6)^2*qd6 - (2310763*qd5*sin(theta6))/1629982 + (63931*qd5)/6519928 - (3261489*qd6)/3259964)*sin(theta3)*qd1*sin(theta4) + 13039856*cos(theta6)^2*qd5*qd6 + (-9243052*qd1^2 + 9243052*qd2^2 + 18486104*qd2*qd3 + 9243052*qd3^2 - 9243052*qd5^2 + 9243052*qd6^2)*sin(theta6) + 63931*qd1^2 - 63931*qd2^2 - 127862*qd2*qd3 - 63931*qd3^2 + 63931*qd5^2 - 13045956*qd5*qd6)*sin(theta5))/1000000000 + 2310763*(qd6*sin(theta6) + (26683037*qd5)/18486104)*(qd2 + qd3)*sin(theta4)/125000000 + (814991*qd1*sin(theta2)*sin(theta3)*(qd2 + qd3)*cos(theta6)^2)/62500000 + ((13039856*sin(theta6)*qd4*qd6 + 18486104*qd4*qd5)*cos(theta6))/1000000000 - (193696127*qd1*sin(theta2)*sin(theta3)*(qd2 + qd3))/1000000000 + (510879*qd1^2)/500000000 - (510879*qd2^2)/500000000 - (510879*qd2*qd3)/250000000 - (510879*qd3^2)/500000000 - (5043*qd4*qd5)/62500000;
v5 = ((-36972208*(cos(theta6) - 10086/2310763)*(qd1^2*(cos(theta3)^2 - 1/2)*cos(theta2)^2 - qd1^2*cos(theta2)*cos(theta3)*sin(theta3)*sin(theta2) - qd1^2*cos(theta3)^2/2 + ((qd1 + qd2 + qd3)*(qd1 - qd2 - qd3))/2)*cos(theta4)^2 - 26079712*qd1*(qd1*cos(theta3)*sin(theta3)*(cos(theta6)^2 + 16011145/6519928)*cos(theta2)^2 + (qd1*sin(theta2)*(cos(theta6)^2 + 16011145/6519928)*cos(theta3)^2 + (qd4*cos(theta6)^2/2 + (2310763*sin(theta4)*(qd2 + qd3)*cos(theta6))/1629982 + (-(5043*qd2)/814991 - (5043*qd3)/814991)*sin(theta4) + (16011145*qd4)/13039856)*cos(theta3) - qd1*sin(theta2)*(cos(theta6)^2 + 16011145/6519928)/2)*cos(theta2) - sin(theta3)*(qd1*(cos(theta6)^2 + 16011145/6519928)*cos(theta3) + (qd4*cos(theta6)^2 + (2310763*sin(theta4)*(qd2 + qd3)*cos(theta6))/814991 + (-(10086*qd2)/814991 - (10086*qd3)/814991)*sin(theta4) + (16011145*qd4)/6519928)*sin(theta2))/2)*cos(theta4) - 36972208*(cos(theta6) - 10086/2310763)*(cos(theta3)^2 - 1/2)*qd1^2*cos(theta2)^2 + 36972208*(qd1*sin(theta2)*(cos(theta6) - 10086/2310763)*cos(theta3) - (814991*sin(theta4)*(qd2 + qd3)*cos(theta6)^2)/2310763 + cos(theta6)*qd4 + (-(16011145*qd2)/18486104 - (16011145*qd3)/18486104)*sin(theta4) - (10086*qd4)/2310763)*sin(theta3)*qd1*cos(theta2) + (18486104*qd1^2*cos(theta6) - 80688*qd1^2)*cos(theta3)^2 - 13039856*(sin(theta4)*(qd2 + qd3)*cos(theta6)^2 - (2310763*cos(theta6)*qd4)/814991 + ((16011145*qd2)/6519928 + (16011145*qd3)/6519928)*sin(theta4) + (10086*qd4)/814991)*sin(theta2)*qd1*cos(theta3) - 13039856*qd4*sin(theta4)*(qd2 + qd3)*cos(theta6)^2 - 18486104*(qd2 + qd3 + qd4)*(qd2 + qd3 - qd4)*cos(theta6) - 32022290*qd4*sin(theta4)*(qd2 + qd3) + 80688*(qd2 + qd3 + qd4)*(qd2 + qd3 - qd4))*cos(theta5)^2)/1000000000 + (((-13039856*sin(theta5)*(cos(theta6)^2 + 16011145/6519928)*qd1^2*(cos(theta3)^2 - 1/2)*cos(theta2)^2 + 13039856*(qd1*cos(theta6)^2*sin(theta2)*sin(theta3)*sin(theta5) + (16011145*qd1*sin(theta2)*sin(theta3)*sin(theta5))/6519928 - 2310763*(-9133/1320436 + sin(theta6))*(qd2 + qd3)/1629982)*qd1*cos(theta3)*cos(theta2) + 6519928*sin(theta5)*(cos(theta6)^2 + 16011145/6519928)*qd1^2*cos(theta3)^2 - 6519928*sin(theta5)*(qd1 + qd2 + qd3)*(qd1 - qd2 - qd3)*cos(theta6)^2 - 16011145*sin(theta5)*(qd1 + qd2 + qd3)*(qd1 - qd2 - qd3) + 18486104*sin(theta2)*(-9133/1320436 + sin(theta6))*sin(theta3)*qd1*(qd2 + qd3))*cos(theta4)^2 + (18486104*(sin(theta4)*(-9133/1320436 + sin(theta6))*cos(theta3)^2 + (4*cos(theta6)*sin(theta3)*sin(theta5) - (40344*sin(theta5)*sin(theta3))/2310763 - (270750*sin(theta3))/2310763 - 128250/2310763)*cos(theta3) - sin(theta4)*(-9133/1320436 + sin(theta6))/2)*qd1^2*cos(theta2)^2 + 73944416*(qd1*sin(theta2)*(sin(theta5)*cos(theta6) - (10086*sin(theta5))/2310763 - 135375/4621526)*cos(theta3)^2 + ((-(814991*sin(theta4)*(qd2 + qd3)*sin(theta5))/4621526 - (814991*qd6)/4621526)*cos(theta6)^2 + cos(theta6)*sin(theta5)*qd4/2 + ((-(16011145*qd2)/36972208 - (16011145*qd3)/36972208)*sin(theta4) - (5043*qd4)/2310763)*sin(theta5) - sin(theta2)*sin(theta3)*qd1*(-9133/1320436 + sin(theta6))*sin(theta4)/4 - (1525*qd6)/18486104)*cos(theta3) - ((sin(theta5)*sin(theta2)*cos(theta6) - (10086*sin(theta5)*sin(theta2))/2310763 + (-(64125*sin(theta2))/2310763 + 7125/1320436)*sin(theta3) - (135375*sin(theta2))/4621526)*qd1)/2)*qd1*cos(theta2) - 9243052*qd1^2*(-9133/1320436 + sin(theta6))*sin(theta4)*cos(theta3)^2 + (-36972208*qd1^2*cos(theta6)*sin(theta3)*sin(theta5) + 161376*qd1^2*sin(theta3)*sin(theta5) - 199500*qd1^2*sin(theta2) + 1083000*qd1^2*sin(theta3) + 1026000*qd1^2 + 1026000*qd2^2)*cos(theta3) + 13039856*sin(theta2)*sin(theta3)*qd1*(sin(theta4)*(qd2 + qd3)*sin(theta5) + qd6)*cos(theta6)^2 - 36972208*qd4*(qd1*sin(theta2)*sin(theta3)*sin(theta5) + (814991*sin(theta6)*(qd2 + qd3))/2310763)*cos(theta6) + 32022290*sin(theta2)*(sin(theta4)*(qd2 + qd3) + (80688*qd4)/16011145)*sin(theta3)*qd1*sin(theta5) + 9243052*(qd1 + qd2 + qd3)*(-9133/1320436 + sin(theta6))*(qd1 - qd2 - qd3)*sin(theta4) + 6100*qd1*sin(theta2)*sin(theta3)*qd6 + 92960178*qd4*(qd2 + qd3))*cos(theta4) - 13039856*(sin(theta5)*(cos(theta6)^2 + 16011145/6519928)*cos(theta3)^2 - sin(theta3)*(cos(theta6)*sin(theta6) - 46480089/6519928)*sin(theta4)*cos(theta3) - sin(theta5)*(cos(theta6)^2 + 16011145/6519928)/2)*qd1^2*cos(theta2)^2 + 13039856*(qd1*sin(theta2)*sin(theta4)*(cos(theta6)*sin(theta6) - 46480089/6519928)*cos(theta3)^2 + (qd1*cos(theta6)^2*sin(theta2)*sin(theta3)*sin(theta5) + cos(theta6)*sin(theta4)*sin(theta6)*qd4 + (16011145*qd1*sin(theta2)*sin(theta3)*sin(theta5))/6519928 - (46480089*qd4*sin(theta4))/6519928 + 2310763*(-9133/1320436 + sin(theta6))*(qd2 + qd3)/1629982)*cos(theta3) + cos(theta6)^2*sin(theta3)*sin(theta5)*qd4 + ((2310763*sin(theta3)*sin(theta4)*(qd2 + qd3)*sin(theta5))/814991 - qd1*sin(theta2)*sin(theta4)*sin(theta6)/2 + (2310763*sin(theta3)*qd6)/1629982)*cos(theta6) - (10086*sin(theta3)*(sin(theta4)*(qd2 + qd3) - (16011145*qd4)/80688)*sin(theta5))/814991 + 46480089*((-(722000*qd2)/15493363 - (722000*qd3)/15493363)*sin(theta3) + qd1*sin(theta2) - (684000*qd2)/15493363)*sin(theta4)/13039856)*qd1*cos(theta2) + 6519928*sin(theta5)*(cos(theta6)^2 + 16011145/6519928)*qd1^2*cos(theta3)^2 - 6519928*qd1*(-2*cos(theta6)^2*sin(theta2)*sin(theta5)*qd4 + (-(4621526*sin(theta2)*sin(theta4)*(qd2 + qd3)*sin(theta5))/814991 + qd1*sin(theta3)*sin(theta4)*sin(theta6) - (2310763*sin(theta2)*qd6)/814991)*cos(theta6) + (20172*sin(theta2)*(sin(theta4)*(qd2 + qd3) - (16011145*qd4)/80688)*sin(theta5))/814991 - 46480089*(qd1*sin(theta3) - (722000*sin(theta2)*(qd2 + qd3))/15493363)*sin(theta4)/6519928)*cos(theta3) + (-6519928*(qd2 + qd3 + qd4)*(qd2 + qd3 - qd4)*sin(theta5) - 13039856*qd6*sin(theta4)*(qd2 + qd3))*cos(theta6)^2 - 13039856*(-(2310763*sin(theta4)*(qd2 + qd3)*sin(theta5))/814991 + qd1*sin(theta2)*sin(theta3)*sin(theta4)*sin(theta6) - (2310763*qd6)/1629982)*qd4*cos(theta6) + (-161376*qd4*sin(theta4)*(qd2 + qd3) - 16011145*(qd2 + qd3 + qd4)*(qd2 + qd3 - qd4))*sin(theta5) + (92960178*qd4*qd1*sin(theta3)*sin(theta2) - 6100*qd6*(qd2 + qd3))*sin(theta4) - 18486104*sin(theta2)*(-9133/1320436 + sin(theta6))*sin(theta3)*qd1*(qd2 + qd3))*cos(theta5))/1000000000 + ((18486104*(cos(theta6) - 10086/2310763)*(cos(theta3)^2 - 1/2)*qd1^2*cos(theta2)^2 - 18486104*(((1629982*sin(theta6)*(qd2 + qd3)*sin(theta5))/2310763 + qd1*sin(theta2)*sin(theta3))*cos(theta6) + (-(46480089*qd2)/9243052 - (46480089*qd3)/9243052)*sin(theta5) - (10086*qd1*sin(theta2)*sin(theta3))/2310763)*qd1*cos(theta3)*cos(theta2) + (-9243052*qd1^2*cos(theta6) + 40344*qd1^2)*cos(theta3)^2 + (13039856*qd1*sin(theta2)*sin(theta3)*sin(theta6)*(qd2 + qd3)*sin(theta5) + 9243052*(qd1 + qd2 + qd3)*(qd1 - qd2 - qd3))*cos(theta6) - 92960178*qd1*sin(theta2)*sin(theta3)*(qd2 + qd3)*sin(theta5) - 40344*(qd1 + qd2 + qd3)*(qd1 - qd2 - qd3))*cos(theta4)^2)/1000000000 + ((13039856*qd1^2*(sin(theta4)*sin(theta5)*(cos(theta6)*sin(theta6) - 46480089/6519928)*cos(theta3)^2 + sin(theta3)*(cos(theta6)^2 + 16011145/6519928)*cos(theta3) - sin(theta4)*sin(theta5)*(cos(theta6)*sin(theta6) - 46480089/6519928)/2)*cos(theta2)^2 + 13039856*(qd1*sin(theta2)*(cos(theta6)^2 + 16011145/6519928)*cos(theta3)^2 + (((-qd1*sin(theta2)*sin(theta3)*sin(theta4)*sin(theta6) + (2310763*qd6)/1629982)*sin(theta5) + (2310763*sin(theta4)*(qd2 + qd3))/1629982)*cos(theta6) + (46480089*qd1*sin(theta2)*sin(theta3)*sin(theta4)*sin(theta5))/6519928 + (-(5043*qd2)/814991 - (5043*qd3)/814991)*sin(theta4) - (26683037*qd4)/13039856)*cos(theta3) - qd1*sin(theta2)*(cos(theta6)^2 + 16011145/6519928)/2)*qd1*cos(theta2) - 6519928*sin(theta5)*qd1^2*sin(theta4)*(cos(theta6)*sin(theta6) - 46480089/6519928)*cos(theta3)^2 - 6519928*(cos(theta6)^2 + 16011145/6519928)*sin(theta3)*qd1^2*cos(theta3) + ((6519928*sin(theta6)*(qd1 + qd2 + qd3)*(qd1 - qd2 - qd3)*sin(theta4) - 18486104*qd1*sin(theta2)*sin(theta3)*qd6)*sin(theta5) - 18486104*(qd1*sin(theta2)*sin(theta3)*sin(theta4) + (1629982*qd6*sin(theta6))/2310763)*(qd2 + qd3))*cos(theta6) + (-46480089*(qd1 + qd2 + qd3)*(qd1 - qd2 - qd3)*sin(theta4) + 18486104*qd4*(-9133/1320436 + sin(theta6))*(qd2 + qd3))*sin(theta5) + 80688*sin(theta2)*(sin(theta4)*(qd2 + qd3) + (26683037*qd4)/80688)*sin(theta3)*qd1)*cos(theta4))/1000000000 + 2310763*((cos(theta6) - (270750*sin(theta5))/2310763 - 10086/2310763)*cos(theta3)^2 - sin(theta5)*(-9133/1320436 + sin(theta6))*sin(theta3)*sin(theta4)*cos(theta3) - cos(theta6)/2 + 5043/2310763 + ((128250*sin(theta3))/2310763 + 135375/2310763)*sin(theta5))*qd1^2*cos(theta2)^2/125000000 - 2310763*(qd1*sin(theta2)*sin(theta4)*sin(theta5)*(-9133/1320436 + sin(theta6))*cos(theta3)^2 + ((-(1629982*sin(theta6)*(qd2 + qd3)*sin(theta5))/2310763 + qd1*sin(theta2)*sin(theta3) - (1629982*sin(theta4)*sin(theta6)*qd6)/2310763)*cos(theta6) + (qd4*(-9133/1320436 + sin(theta6))*sin(theta4) - (270750*qd1*sin(theta2)*sin(theta3))/2310763 - (128250*qd1*sin(theta2))/2310763 + (7125*qd1)/660218 + (46480089*qd2)/9243052 + (46480089*qd3)/9243052)*sin(theta5) - (10086*qd1*sin(theta2)*sin(theta3))/2310763)*cos(theta3) - 1629982*(sin(theta5)*qd6 + sin(theta4)*(qd2 + qd3))*sin(theta3)*cos(theta6)^2/2310763 + cos(theta6)*sin(theta3)*qd4 + (-sin(theta2)*(-9133/1320436 + sin(theta6))*qd1*sin(theta4)/2 - (1525*sin(theta3)*qd6)/4621526)*sin(theta5) - (58705327*sin(theta3)*(sin(theta4)*(qd2 + qd3) + (80688*qd4)/58705327))/18486104)*qd1*cos(theta2)/125000000 + ((-9243052*qd1^2*cos(theta6) + 1083000*qd1^2*sin(theta5) + 40344*qd1^2)*cos(theta3)^2)/1000000000 + (2310763*qd1*((3259964*sin(theta2)*(sin(theta5)*qd6 + sin(theta4)*(qd2 + qd3))*cos(theta6)^2)/2310763 - 2*cos(theta6)*sin(theta2)*qd4 + (qd1*sin(theta3)*(-9133/1320436 + sin(theta6))*sin(theta4) + (1525*sin(theta2)*qd6)/2310763)*sin(theta5) + (58705327*sin(theta2)*(sin(theta4)*(qd2 + qd3) + (80688*qd4)/58705327))/9243052)*cos(theta3))/250000000 + (814991*cos(theta6)^2*sin(theta5)*qd4*qd6)/62500000 + ((-13039856*(qd1*sin(theta2)*sin(theta3)*sin(theta6) - (2310763*qd6*sin(theta4))/1629982)*(qd2 + qd3)*sin(theta5) - 13039856*qd1*sin(theta2)*sin(theta3)*sin(theta4)*sin(theta6)*qd6 - 13039856*sin(theta6)*qd5*qd6 + 9243052*qd2^2 + 18486104*qd2*qd3 + 9243052*qd3^2 - 9243052*qd4^2 + 9243052*qd6^2)*cos(theta6))/1000000000 + ((18486104*sin(theta2)*(-9133/1320436 + sin(theta6))*qd4*sin(theta3)*qd1*sin(theta4) + (199500*(qd1 + (15493363*qd2)/33250 + (15493363*qd3)/33250)*qd1*sin(theta2) - 1026000*qd1^2 - 1026000*qd2^2)*sin(theta3) - 1083000*qd1^2 - 1083000*qd2^2 - 2166000*qd2*qd3 - 1083000*qd3^2 + 6100*qd4*qd6)*sin(theta5))/1000000000 - (26683037*qd4*sin(theta4)*(qd2 + qd3))/1000000000 - 5043*(qd2 + qd3 + qd4)*(qd2 + qd3 - qd4)/125000000;
v6 = (((6519928*qd1*(qd2 + qd3)*(cos(theta2)*cos(theta3) - sin(theta2)*sin(theta3))*cos(theta4)^2 + (-6519928*sin(theta4)*qd1^2*(cos(theta3)^2 - 1/2)*cos(theta2)^2 + 6519928*qd1*(qd1*sin(theta2)*sin(theta3)*sin(theta4) + qd5/2)*cos(theta3)*cos(theta2) + 3259964*qd1^2*cos(theta3)^2*sin(theta4) - 3259964*(qd1 + qd2 + qd3)*(qd1 - qd2 - qd3)*sin(theta4) - 3259964*qd1*sin(theta2)*sin(theta3)*qd5)*cos(theta4) - 3259964*(qd2 + qd3)*(qd1*cos(theta2)*cos(theta3) - qd1*sin(theta2)*sin(theta3) - qd5*sin(theta4)))*cos(theta5) + 6519928*(-((qd2 + qd3)*(qd1*cos(theta2)*sin(theta3) + qd1*cos(theta3)*sin(theta2) + qd4)*cos(theta4))/2 + qd1^2*cos(theta2)^2*cos(theta3)*sin(theta3)*sin(theta4) + qd1*(qd1*cos(theta3)^2*sin(theta2)*sin(theta4) - qd1*sin(theta2)*sin(theta4)/2 + cos(theta3)*sin(theta4)*qd4/2 - sin(theta3)*qd5/2)*cos(theta2) - qd1*(qd1*sin(theta3)*sin(theta4) + qd5*sin(theta2))*cos(theta3)/2 - qd4*(qd1*sin(theta2)*sin(theta3)*sin(theta4) + qd5)/2)*sin(theta5))*cos(theta6)^2)/250000000 + ((-3259964*sin(theta6)*((qd1^2*(cos(theta3)^2 - 1/2)*cos(theta2)^2 - qd1^2*cos(theta2)*cos(theta3)*sin(theta3)*sin(theta2) - qd1^2*cos(theta3)^2/2 + ((qd1 + qd2 + qd3)*(qd1 - qd2 - qd3))/2)*cos(theta4)^2 + qd1*sin(theta4)*(qd2 + qd3)*(cos(theta2)*cos(theta3) - sin(theta2)*sin(theta3))*cos(theta4) + qd1^2*(cos(theta3)^2 - 1/2)*cos(theta2)^2 - qd1*sin(theta3)*(qd1*cos(theta3)*sin(theta2) + qd4)*cos(theta2) - qd1^2*cos(theta3)^2/2 - qd1*cos(theta3)*sin(theta2)*qd4 + ((qd2 + qd3 + qd4)*(qd2 + qd3 - qd4))/2)*cos(theta5)^2 + (6519928*qd1*((qd1*cos(theta2)^2*cos(theta3)*sin(theta3) + (qd1*cos(theta3)^2*sin(theta2) - qd1*sin(theta2)/2 + cos(theta3)*qd4/2)*cos(theta2) - sin(theta3)*(qd1*cos(theta3) + sin(theta2)*qd4)/2)*sin(theta5)*sin(theta6) - 2310763*(qd2 + qd3)*(cos(theta2)*sin(theta3) + sin(theta2)*cos(theta3))/3259964)*cos(theta4) + 3259964*sin(theta4)*sin(theta5)*(qd2 + qd3)*(qd1*cos(theta2)*sin(theta3) + qd1*cos(theta3)*sin(theta2) + qd4)*sin(theta6) + 4621526*qd1^2*cos(theta2)^2*cos(theta3)*sin(theta3)*sin(theta4) + 4621526*(qd1*cos(theta3)^2*sin(theta2)*sin(theta4) - qd1*sin(theta2)*sin(theta4)/2 - sin(theta3)*qd5)*qd1*cos(theta2) - 2310763*qd1*(qd1*sin(theta3)*sin(theta4) + 2*qd5*sin(theta2))*cos(theta3) - 4621526*qd4*qd5)*cos(theta5) + ((-3259964*qd1^2*(cos(theta3)^2 - 1/2)*cos(theta2)^2 + 3259964*qd1^2*cos(theta2)*cos(theta3)*sin(theta3)*sin(theta2) + 1629982*qd1^2*cos(theta3)^2 - 1629982*(qd1 + qd2 + qd3)*(qd1 - qd2 - qd3))*sin(theta6) - 4621526*qd1*sin(theta5)*(qd2 + qd3)*(cos(theta2)*cos(theta3) - sin(theta2)*sin(theta3)))*cos(theta4)^2 + (-3259964*(qd2 + qd3)*(qd1*cos(theta2)*cos(theta3)*sin(theta4) - qd1*sin(theta2)*sin(theta3)*sin(theta4) - qd5)*sin(theta6) + 4621526*(sin(theta4)*qd1^2*(cos(theta3)^2 - 1/2)*cos(theta2)^2 - qd1*cos(theta3)*(qd1*sin(theta2)*sin(theta3)*sin(theta4) + qd5)*cos(theta2) - qd1^2*cos(theta3)^2*sin(theta4)/2 + ((qd1 + qd2 + qd3)*(qd1 - qd2 - qd3)*sin(theta4))/2 + qd1*sin(theta2)*sin(theta3)*qd5)*sin(theta5))*cos(theta4) + (6519928*qd1^2*(cos(theta3)^2 - 1/2)*cos(theta2)^2 - 6519928*qd1*((qd1*sin(theta2)*sin(theta3) + qd5*sin(theta4)/2)*cos(theta3) + sin(theta3)*qd4/2)*cos(theta2) + 3259964*qd1*sin(theta2)*sin(theta3)*sin(theta4)*qd5 - 3259964*qd1^2*cos(theta3)^2 - 3259964*qd1*cos(theta3)*sin(theta2)*qd4 + 1629982*qd1^2 - 1629982*qd4^2 + 1629982*qd5^2)*sin(theta6) - 4621526*sin(theta4)*sin(theta5)*qd5*(qd2 + qd3))*cos(theta6))/250000000 + (2310763*sin(theta6)*((qd1*cos(theta2)^2*cos(theta3)*sin(theta3) + (qd1*cos(theta3)^2*sin(theta2) - qd1*sin(theta2)/2 + cos(theta3)*qd4/2)*cos(theta2) - sin(theta3)*(qd1*cos(theta3) + sin(theta2)*qd4)/2)*qd1*cos(theta4) + sin(theta4)*(qd2 + qd3)*(qd1*cos(theta2)*sin(theta3) + qd1*cos(theta3)*sin(theta2) + qd4)/2)*cos(theta5)^2)/62500000 + (((4621526*(qd1^2*(cos(theta3)^2 - 1/2)*cos(theta2)^2 - qd1^2*cos(theta2)*cos(theta3)*sin(theta3)*sin(theta2) - qd1^2*cos(theta3)^2/2 + ((qd1 + qd2 + qd3)*(qd1 - qd2 - qd3))/2)*sin(theta5)*sin(theta6) - 3259964*qd1*(qd2 + qd3)*(cos(theta2)*cos(theta3) - sin(theta2)*sin(theta3)))*cos(theta4)^2 + (4621526*qd1*sin(theta4)*sin(theta5)*(qd2 + qd3)*(cos(theta2)*cos(theta3) - sin(theta2)*sin(theta3))*sin(theta6) + 3259964*sin(theta4)*qd1^2*(cos(theta3)^2 - 1/2)*cos(theta2)^2 - 3259964*qd1*cos(theta3)*(qd1*sin(theta2)*sin(theta3)*sin(theta4) - (1525*qd5)/3259964)*cos(theta2) - 1629982*qd1^2*cos(theta3)^2*sin(theta4) + 1629982*(qd1 + qd2 + qd3)*(qd1 - qd2 - qd3)*sin(theta4) - 1525*qd1*sin(theta2)*sin(theta3)*qd5)*cos(theta4) + 4621526*sin(theta5)*(qd1^2*(cos(theta3)^2 - 1/2)*cos(theta2)^2 - qd1*sin(theta3)*(qd1*cos(theta3)*sin(theta2) + qd4)*cos(theta2) - qd1^2*cos(theta3)^2/2 - qd1*cos(theta3)*sin(theta2)*qd4 + ((qd2 + qd3 + qd4)*(qd2 + qd3 - qd4))/2)*sin(theta6) + 3261489*(qd1*cos(theta2)*cos(theta3) - qd1*sin(theta2)*sin(theta3) + (1525*qd5*sin(theta4))/3261489)*(qd2 + qd3))*cos(theta5))/250000000 + ((-4621526*qd1*(qd1*cos(theta2)^2*cos(theta3)*sin(theta3) + (qd1*cos(theta3)^2*sin(theta2) - qd1*sin(theta2)/2 + cos(theta3)*qd4)*cos(theta2) - sin(theta3)*(qd1*cos(theta3) + 2*sin(theta2)*qd4)/2)*sin(theta6) - 1525*(qd1*cos(theta2)*sin(theta3) + qd1*cos(theta3)*sin(theta2) - (3261489*qd4)/1525)*sin(theta5)*(qd2 + qd3))*cos(theta4))/250000000 - (2310763*sin(theta4)*qd4*(qd2 + qd3)*sin(theta6))/125000000 - (814991*(qd1^2*cos(theta2)^2*cos(theta3)*sin(theta3)*sin(theta4) + qd1*(qd1*cos(theta3)^2*sin(theta2)*sin(theta4) - qd1*sin(theta2)*sin(theta4)/2 + (3261489*cos(theta3)*sin(theta4)*qd4)/3259964 + (1525*sin(theta3)*qd5)/3259964)*cos(theta2) + (-qd1^2*sin(theta3)*sin(theta4)/2 + (1525*qd1*sin(theta2)*qd5)/3259964)*cos(theta3) - 3261489*(qd1*sin(theta2)*sin(theta3)*sin(theta4) - (1525*qd5)/3261489)*qd4/3259964)*sin(theta5))/62500000;

V = [v1; v2; v3; v4; v5; v6];

thetadd = pinv(D) * (u - V - G);

% j1 = [ 65*cos(theta1)*sin(theta4)*sin(theta5) - 65*sin(theta1)*(cos(theta2 + theta3)*cos(theta5) - sin(theta2 + theta3)*cos(theta4)*sin(theta5)) - 70*sin(theta1) + sin(theta1)*sin(theta2)*(380*sin(theta3) + 360) - 380*cos(theta2)*cos(theta3)*sin(theta1), -cos(theta1)*(360*cos(theta2) + 380*cos(theta2)*sin(theta3) + 380*cos(theta3)*sin(theta2) + 65*sin(theta2 + theta3)*cos(theta5) + 65*cos(theta2 + theta3)*cos(theta4)*sin(theta5)), -cos(theta1)*(380*cos(theta3)*sin(theta2) - 360*cos(theta2) + cos(theta5)*(65*cos(theta2)*sin(theta3) + 65*cos(theta3)*sin(theta2)) + cos(theta2)*(380*sin(theta3) + 360) + 65*cos(theta4)*sin(theta5)*(cos(theta2)*cos(theta3) - sin(theta2)*sin(theta3))), 65*sin(theta5)*(cos(theta4)*sin(theta1) + cos(theta1)*cos(theta2)*sin(theta3)*sin(theta4) + cos(theta1)*cos(theta3)*sin(theta2)*sin(theta4)), 65*cos(theta5)*sin(theta1)*sin(theta4) - 65*cos(theta1)*cos(theta2)*cos(theta3)*sin(theta5) + 65*cos(theta1)*sin(theta2)*sin(theta3)*sin(theta5) - 65*cos(theta1)*cos(theta2)*cos(theta4)*cos(theta5)*sin(theta3) - 65*cos(theta1)*cos(theta3)*cos(theta4)*cos(theta5)*sin(theta2), 0];
% j2 = [ cos(theta1)*(65*cos(theta2 + theta3)*cos(theta5) - 65*sin(theta2 + theta3)*cos(theta4)*sin(theta5)) + 10*cos(theta1)*(38*cos(theta2 + theta3) - 36*sin(theta2) + 7) + 65*sin(theta1)*sin(theta4)*sin(theta5), -sin(theta1)*(360*cos(theta2) + 380*cos(theta2)*sin(theta3) + 380*cos(theta3)*sin(theta2) + 65*sin(theta2 + theta3)*cos(theta5) + 65*cos(theta2 + theta3)*cos(theta4)*sin(theta5)), -sin(theta1)*(380*cos(theta3)*sin(theta2) - 360*cos(theta2) + cos(theta5)*(65*cos(theta2)*sin(theta3) + 65*cos(theta3)*sin(theta2)) + cos(theta2)*(380*sin(theta3) + 360) + 65*cos(theta4)*sin(theta5)*(cos(theta2)*cos(theta3) - sin(theta2)*sin(theta3))), 65*sin(theta5)*(cos(theta2)*sin(theta1)*sin(theta3)*sin(theta4) - cos(theta1)*cos(theta4) + cos(theta3)*sin(theta1)*sin(theta2)*sin(theta4)), 65*sin(theta1)*sin(theta2)*sin(theta3)*sin(theta5) - 65*cos(theta2)*cos(theta3)*sin(theta1)*sin(theta5) - 65*cos(theta1)*cos(theta5)*sin(theta4) - 65*cos(theta2)*cos(theta4)*cos(theta5)*sin(theta1)*sin(theta3) - 65*cos(theta3)*cos(theta4)*cos(theta5)*sin(theta1)*sin(theta2), 0];
% j3 = [ 0, 380*cos(theta2)*cos(theta3) - 360*sin(theta2) - 380*sin(theta2)*sin(theta3) - 65*cos(theta5)*sin(theta2)*sin(theta3) + 65*cos(theta2)*cos(theta3)*cos(theta5) - 65*cos(theta2)*cos(theta4)*sin(theta3)*sin(theta5) - 65*cos(theta3)*cos(theta4)*sin(theta2)*sin(theta5), 380*cos(theta2)*cos(theta3) - 380*sin(theta2)*sin(theta3) - 65*cos(theta5)*sin(theta2)*sin(theta3) + 65*cos(theta2)*cos(theta3)*cos(theta5) - 65*cos(theta2)*cos(theta4)*sin(theta3)*sin(theta5) - 65*cos(theta3)*cos(theta4)*sin(theta2)*sin(theta5), -65*cos(theta2 + theta3)*sin(theta4)*sin(theta5), 65*cos(theta2)*cos(theta3)*cos(theta4)*cos(theta5) - 65*cos(theta3)*sin(theta2)*sin(theta5) - 65*cos(theta2)*sin(theta3)*sin(theta5) - 65*cos(theta4)*cos(theta5)*sin(theta2)*sin(theta3), 0];
% j4 = [ 0, sin(theta1), sin(theta1), cos(theta2 + theta3)*cos(theta1), cos(theta4)*sin(theta1) + cos(theta1)*sin(theta4)*(cos(theta2)*sin(theta3) + cos(theta3)*sin(theta2)), cos(theta1)*(cos(theta2 + theta3)*cos(theta5) - sin(theta2 + theta3)*cos(theta4)*sin(theta5)) + sin(theta1)*sin(theta4)*sin(theta5)];
% j5 = [ 0, -cos(theta1), -cos(theta1), cos(theta2 + theta3)*sin(theta1), sin(theta1)*sin(theta4)*(cos(theta2)*sin(theta3) + cos(theta3)*sin(theta2)) - cos(theta1)*cos(theta4), sin(theta1)*(cos(theta2 + theta3)*cos(theta5) - sin(theta2 + theta3)*cos(theta4)*sin(theta5)) - cos(theta1)*sin(theta4)*sin(theta5)];
% j6 = [ 1, 0, 0, sin(theta2 + theta3), -cos(theta2 + theta3)*sin(theta4), sin(theta2 + theta3)*cos(theta5) + cos(theta2 + theta3)*cos(theta4)*sin(theta5)];
% 
% J = [j1; j2; j3; j4; j5; j6];

% Dx = transpose(pinv(J))*D*pinv(J);
% Vx = transpose(pinv(J))*V;
% Gx = transpose(pinv(J))*G;
% 
% xdd = pinv(Dx)*(u - Vx - Gx);
